simulink model "IEEE123bus_v2019b_Phasor_PI_ZIPload"  (R2019b)
settings: Solver=ode4  StartTime=0.0  StopTime=100  FixedStep=Ts  MaxStep=1e-4  RelTol=1e-3
InitFcn:
  | a=1; % Loading Factor
  | Ts=0.1;% For Delay Blocks in Voltage Regulator Controls
  | % phase to sequence conversion of RXB matrices
  | c=1*exp(sqrt(-1)*(120*pi/180));
  | T=[1 1 1;1 c*c c;1 c c*c];
  | Tinv=1/3*[1 1 1;1 c c*c;1 c*c c];
  | 
  | % Simulation data for the IEEE 123 Node Test Feeder model
  | mi2km = 1.60934;%  miles to km conversion
  | ft2km = 0.0003048; % feet to km conversion
  | ms2F = 1*1e-6/(2*pi*60);% microsiemens to Farads conversion
  | 
  | %% Configuration 1
  | % Series Resitance and Reactance - ohm/mile
  | R_1 = [0.4576 0.1560 0.1535;0.1560 0.4666 0.1580;0.1535 0.1580 0.4615];
  | X_1 = [1.0780 0.5017 0.3849;0.5017 1.0482 0.4236;0.3849 0.4236 1.0651];
  | % charging susceptance - microsiemens/mile
  | B_1 = [5.6765 -1.8319 -0.6982;-1.8319 5.9809 -1.1645;-0.6982 -1.1645 5.3971];
  | 
  | R_1 = R_1/mi2km;
  | Rseq=Tinv*R_1*T;
  | R1_1=Rseq(2,2);R0_1=Rseq(1,1);
  | 
  | L_1 = (X_1/(2*pi*60))/mi2km;
  | Lseq=Tinv*L_1*T;
  | L1_1=Lseq(2,2);L0_1=Lseq(1,1);
  | 
  | C_1 =(B_1*ms2F)/mi2km;
  | Cseq=Tinv*C_1*T;
  | C1_1=Cseq(2,2);C0_1=Cseq(1,1);
  | %% Configuration 2 - series reactance - ohm/mile
  | R_2 = [0.4666 0.1580 0.1560;0.1580 0.4615 0.1535;0.1560 0.1535 0.4576];
  | X_2 = [1.0482 0.4236 0.5017;0.4236 1.0651 0.3849;0.5017 0.3849 1.0780];
  | % charging susceptance - microsiemens/mile
  | B_2 = [5.9809 -1.1645 -1.8319;-1.1645 5.3971 -0.6982;-1.8319 -0.6982 5.6765];
  | 
  | R_2 = R_2/mi2km;
  | Rseq=Tinv*R_2*T;
  | R1_2=Rseq(2,2);R0_2=Rseq(1,1);
  | 
  | L_2 = (X_2/(2*pi*60))/mi2km;
  | Lseq=Tinv*L_2*T;
  | L1_2=Lseq(2,2);L0_2=Lseq(1,1);
  | 
  | C_2 =(B_2*ms2F)/mi2km;
  | Cseq=Tinv*C_2*T;
  | C1_2=Cseq(2,2);C0_2=Cseq(1,1);
  | %% Configuration 3 - series reactance - ohm/mile
  | R_3 = [0.4615 0.1535 0.1580;0.1535 0.4576 0.1560;0.1580 0.1560 0.4666];
  | X_3 = [1.0651 0.3849 0.4236;0.3849 1.0780 0.5017;0.4236 0.5017 1.0482];
  | % charging susceptance - microsiemens/mile
  | B_3 = [5.3971 -0.6982 -1.1645;-0.6982 5.6765 -1.8319; -1.1645 -1.8319 5.9809];
  | 
  | R_3 = R_3/mi2km;
  | Rseq=Tinv*R_3*T;
  | R1_3=Rseq(2,2);R0_3=Rseq(1,1);
  | 
  | L_3 = (X_3/(2*pi*60))/mi2km;
  | Lseq=Tinv*L_3*T;
  | L1_3=Lseq(2,2);L0_3=Lseq(1,1);
  | 
  | C_3 =(B_3*ms2F)/mi2km;
  | Cseq=Tinv*C_3*T;
  | C1_3=Cseq(2,2);C0_3=Cseq(1,1);
  | %% Configuration 4 - series reactance - ohm/mile
  | R_4 = [0.4615 0.1580 0.1535;0.1580 0.4666 0.1560;0.1535 0.1560 0.4576];
  | X_4 = [1.0651 0.4236 0.3849;0.4236 1.0482 0.5017;0.3849 0.5017 1.0780];
  | % charging susceptance - microsiemens/mile
  | B_4 = [5.3971 -1.1645 -0.6982;-1.1645 5.9809 -1.8319;-0.6982 -1.8319 5.6765];
  | 
  | R_4 = R_4/mi2km;
  | Rseq=Tinv*R_4*T;
  | R1_4=Rseq(2,2);R0_4=Rseq(1,1);
  | 
  | L_4 = (X_4/(2*pi*60))/mi2km;
  | Lseq=Tinv*L_4*T;
  | L1_4=Lseq(2,2);L0_4=Lseq(1,1);
  | 
  | C_4 =(B_4*ms2F)/mi2km;
  | Cseq=Tinv*C_4*T;
  | C1_4=Cseq(2,2);C0_4=Cseq(1,1);
  | %% Configuration 5 - series reactance - ohm/mile
  | R_5 = [0.4666 0.1560 0.1580;0.1560 0.4576 0.1535;0.1580 0.1535 0.4615];
  | X_5 = [1.0482 0.5017 0.4236;0.5017 1.0780 0.3849;0.4236 0.3849 1.0651];
  | % charging susceptance - microsiemens/mile
  | B_5 = [5.9809 -1.8319 -1.1645;-1.8319 5.6765 -0.6982;-1.1645 -0.6982 5.3971];
  | 
  | R_5 = R_5/mi2km;
  | Rseq=Tinv*R_5*T;
  | R1_5=Rseq(2,2);R0_5=Rseq(1,1);
  | 
  | L_5 = (X_5/(2*pi*60))/mi2km;
  | Lseq=Tinv*L_5*T;
  | L1_5=Lseq(2,2);L0_5=Lseq(1,1);
  | 
  | C_5 =(B_5*ms2F)/mi2km;
  | Cseq=Tinv*C_5*T;
  | C1_5=Cseq(2,2);C0_5=Cseq(1,1);
  | %% Configuration 6 - series reactance - ohm/mile
  | R_6 = [0.4576 0.1535 0.1560;0.1535 0.4615 0.1580;0.1560 0.1580 0.4666];
  | X_6 = [1.0780 0.3849 0.5017;0.3849 1.0651 0.4236;0.5017 0.4236 1.0482];
  | % charging susceptance - microsiemens/mile
  | B_6 = [5.6765 -0.6982 -1.8319;-0.6982 5.3971 -1.1645;-1.8319 -1.1645 5.9809];
  | 
  | R_6 = R_6/mi2km;
  | Rseq=Tinv*R_6*T;
  | R1_6=Rseq(2,2);R0_6=Rseq(1,1);
  | 
  | L_6 = (X_6/(2*pi*60))/mi2km;
  | Lseq=Tinv*L_6*T;
  | L1_6=Lseq(2,2);L0_6=Lseq(1,1);
  | 
  | C_6 =(B_6*ms2F)/mi2km;
  | Cseq=Tinv*C_6*T;
  | C1_6=Cseq(2,2);C0_6=Cseq(1,1);
  | %% Configuration 7 - series reactance - ohm/mile
  | R_7 = [0.4576 0.0000 0.1535;0.0000 0.0000 0.0000;0.1535 0.0000 0.4615];
  | X_7 = [1.0780 0.0000 0.3849;0.0000 0.0000 0.0000;0.3849 0.0000 1.0651];
  | % charging susceptance - microsiemens/mile
  | B_7 = [5.1154 0.0000 -1.0549;0.0000 0.0000 0.0000;-1.0549 0.0000 5.1704];
  | 
  | R_7 = R_7/mi2km;
  | Rseq=Tinv*R_7*T;
  | R1_7=Rseq(2,2);R0_7=Rseq(1,1);
  | 
  | L_7 = (X_7/(2*pi*60))/mi2km;
  | Lseq=Tinv*L_7*T;
  | L1_7=Lseq(2,2);L0_7=Lseq(1,1);
  | 
  | C_7 =(B_7*ms2F)/mi2km;
  | Cseq=Tinv*C_7*T;
  | C1_7=Cseq(2,2);C0_7=Cseq(1,1);
  | %% Configuration 8 - series reactance - ohm/mile
  | R_8 = [0.4576 0.1535 0.0000;0.1535 0.4615 0.0000;0.0000 0.0000 0.0000];
  | X_8 = [1.0780 0.3849 0.0000;0.3849 1.0651 0.0000;0.0000 0.0000 0.0000];
  | % charging susceptance - microsiemens/mile
  | B_8 = [5.1154 -1.0549 0.0000;-1.0549 5.1704 0.0000;0.0000 0.0000 0.0000];
  | 
  | R_8 = R_8/mi2km;
  | Rseq=Tinv*R_8*T;
  | R1_8=Rseq(2,2);R0_8=Rseq(1,1);
  | 
  | L_8 = (X_8/(2*pi*60))/mi2km;
  | Lseq=Tinv*L_8*T;
  | L1_8=Lseq(2,2);L0_8=Lseq(1,1);
  | 
  | C_8 =(B_8*ms2F)/mi2km;
  | Cseq=Tinv*C_8*T;
  | C1_8=Cseq(2,2);C0_8=Cseq(1,1);
  | %% Configuration 9 - series reactance - ohm/mile
  | R_9 = [1.3292 0 0;0 0 0;0 0 0];
  | X_9 = [1.3475 0 0;0 0 0;0 0 0];
  | % charging susceptance - microsiemens/mile
  | B_9 = [4.5193 0 0;0 0 0;0 0 0];
  | 
  | R_9 = R_9/mi2km;
  | Rseq=Tinv*R_9*T;
  | R1_9=Rseq(2,2);R0_9=Rseq(1,1);
  | 
  | L_9 = (X_9/(2*pi*60))/mi2km;
  | Lseq=Tinv*L_9*T;
  | L1_9=Lseq(2,2);L0_9=Lseq(1,1);
  | 
  | C_9 =(B_9*ms2F)/mi2km;
  | Cseq=Tinv*C_9*T;
  | C1_9=Cseq(2,2);C0_9=Cseq(1,1);
  | %% Configuration 10- series reactance - ohm/mile
  | R_10 = [0 0 0;0 1.3292 0;0 0 0];
  | X_10 = [0 0 0;0 1.3475 0;0 0 0];
  | % charging susceptance - microsiemens/mile
  | B_10 = [0 0 0;0 4.5193 0;0 0 0];
  | 
  | R_10 = R_10/mi2km;
  | Rseq=Tinv*R_10*T;
  | R1_10=Rseq(2,2);R0_10=Rseq(1,1);
  | 
  | L_10 = (X_10/(2*pi*60))/mi2km;
  | Lseq=Tinv*L_10*T;
  | L1_10=Lseq(2,2);L0_10=Lseq(1,1);
  | 
  | C_10 =(B_10*ms2F)/mi2km;
  | Cseq=Tinv*C_10*T;
  | C1_10=Cseq(2,2);C0_10=Cseq(1,1);
  | %% Configuration 11 - series reactance - ohm/mile
  | R_11 = [0 0 0;0 0 0;0 0 1.3292];
  | X_11 = [0 0 0;0 0 0;0 0 1.3475];
  | % charging susceptance - microsiemens/mile
  | B_11 = [0 0 0;0 0 0;0 0 4.5193];
  | 
  | R_11 = R_11/mi2km;
  | Rseq=Tinv*R_11*T;
  | R1_11=Rseq(2,2);R0_11=Rseq(1,1);
  | 
  | L_11 = (X_11/(2*pi*60))/mi2km;
  | Lseq=Tinv*L_11*T;
  | L1_11=Lseq(2,2);L0_11=Lseq(1,1);
  | 
  | C_11 =(B_11*ms2F)/mi2km;
  | Cseq=Tinv*C_11*T;
  | C1_11=Cseq(2,2);C0_11=Cseq(1,1);
  | %% Configuration 12 - series reactance - ohm/mile
  | R_12 = [1.5209 0.5198 0.4924;0.5198 1.5329 0.5198;0.4924 0.5198 1.5209];
  | X_12 = [0.7521 0.2775 0.2157;0.2775 0.7162 0.2775;0.2157 0.2775 0.7521];
  | % charging susceptance - microsiemens/mile
  | B_12 = [67.2242 0.0000 0.0000;0.0000 67.2242 0.0000;0.0000 0.0000 67.2242];
  | 
  | R_12 = R_12/mi2km;
  | Rseq=Tinv*R_12*T;
  | R1_12=Rseq(2,2);R0_12=Rseq(1,1);
  | 
  | L_12 = (X_12/(2*pi*60))/mi2km;
  | Lseq=Tinv*L_12*T;
  | L1_12=Lseq(2,2);L0_12=Lseq(1,1);
  | 
  | C_12 =(B_12*ms2F)/mi2km;
  | Cseq=Tinv*C_12*T;
  | C1_12=Cseq(2,2);C0_12=Cseq(1,1);
undefined symbols (not defined in the file or in its folder): D1, Delta, find_system, j
libraries: powerlib x974, powerlib_meascontrol x31
(part 1 of 13)
settings Model: ARTEMISmethode_block_infos=$$__separator__$$pi123variableloadwith3PV/ARTEMIS Guide$$__separator__$$  Creator=Arun  LastModifiedBy=USARSUR
settings DataIOCC: ReturnWorkspaceOutputs=off
settings DebuggingCC: UnconnectedInputMsg=none  UnconnectedOutputMsg=none  UnconnectedLineMsg=none  ArithmeticOperatorsInVariantConditions=warning
settings SFSimCC: SimUseLocalCustomCode=off  CustomCodeUndefinedFunction=UseInterfaceOnly
settings RTWCC: RTWUseLocalCustomCode=off
settings CodeAppCC: StateflowObjectComments=on
settings SimscapeCC: SimscapeNormalizeSystem=off

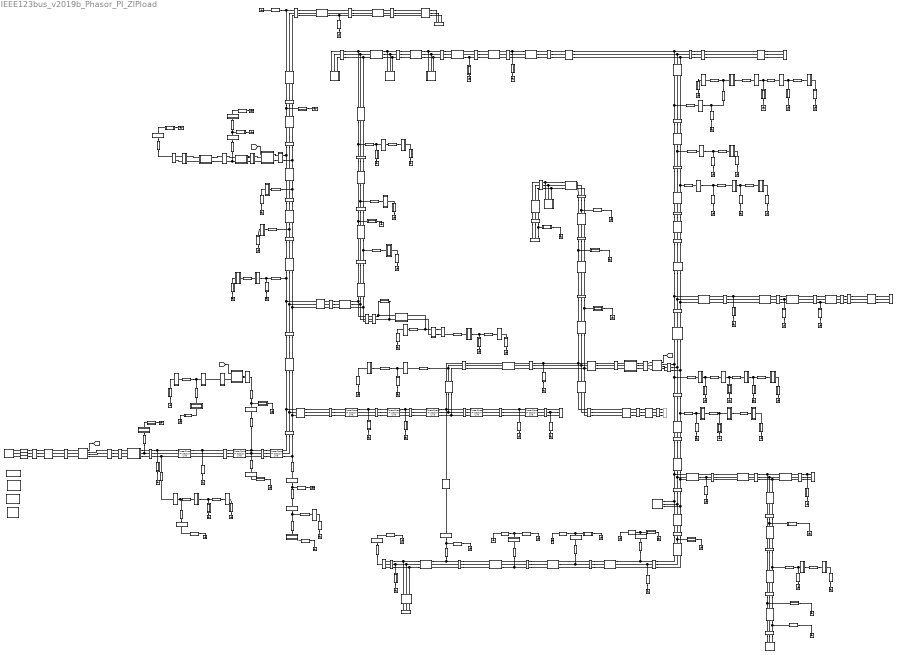
== system IEEE123bus_v2019b_Phasor_PI_ZIPload ==
  note: Please consider citing following papers if the model was useful for your research
      |
      | A. Suresh, R. Bisht and S. Kamalasadan, "A Coordinated Control Architecture With Inverter-Based Resources and Legacy
      | Controllers of Power Distribution System for Voltage Profile Balance," in IEEE Transactions on Industry Applications, vol. 58,
      | no. 5, pp. 6701-6712, Sept.-Oct. 2022, doi: 10.1109/TIA.2022.3183030.
      |
      | A. Suresh, R. Bisht and S. Kamalasadan, "ADMM Based LQR for Voltage Regulation Using Distributed Energy Resources,"
      | 2020 IEEE International Conference on Power Electronics, Drives and Energy Systems (PEDES), 2020, pp. 1-6,
      | doi: 10.1109/PEDES49360.2020.9379625.
  note: Model Developed by
      | Arun Suresh, Dr. Sukumar Kamalasadan,
      | University of North Carolina, Charlotte
  1 : powerlib/Measurements/Three-Phase V-I Measurement  VoltageMeasurement=phase-to-ground  SetLabelV=on  LabelV=V1  Vpu=off  VpuLL=off  CurrentMeasurement=no  SetLabelI=on  LabelI=I800  Ipu=off  Pbase=100e6  Vbase=24900  OutputType=Complex  PhasorSimulation=on  PSBequivalent=0
      settings: SourceProductName=Simscape Electrical
  1 Y PQ : Subsystem  mask(Single Phase ZIP Load){Vnom=1.0*2401.78, fnom=60, Pnom=40e3*a, Qnom=20e3*a, LoadType=constant P, Vlim=0.7}
      mask prompts: Vnom "Nominal Voltage Vn (Vrms)"; fnom "Nominal Frequency fn (Hz)"; Pnom "Nominal Active power (W)"; Qnom "Nominal Reactive power (VAR)"; LoadType "Load Type"; Vlim "Minimum voltage (pu)"
      mask help:
      | Notes:
      | Single Phase ZIP load model which gets converted to constant Z type if the voltage becomes lower than the Minimum Voltage.
      mask TypeOptions LoadType: Constant Z | constant I | constant P
      mask DialogControl ParameterTabVar0 Prompt: Parameters
      mask DialogControl ParameterTabVar1 Prompt: Type
      mask Display:
      | color('red');
      | A=[-210,-180,-170,-160,-147,-140,-130,-120,-110,-80,-50,-49,-45,-39,-33,-26,-21,-18,-17,-19,-22,-22,-26,-27,-25,-22,-16,-9,-3,2,6,6,4,1,1,-3,-4,-2,2,7,14,20,26,29,30,28,24,24,21,20,21,25,31,37,44,49,50,50,80];
      | B=[-41.5,-41.5,-63,-20,-63,-20,-63,-20,-41.5,-41.5,-41.5,-34,-26,-21,-20,-22,-28,-37,-47,-57,-63,-63,-54,-44,-34,-26,-21,-20,-22,-28,-37,-47,-57,-63,-63,-54,-44,-34,-26,-21,-20,-22,-28,-37,-47,-57,-63,-63,-54,-44,-34,-26,-21,-20,-22,-28,-37,-41.50,-41.5];
      | plot(A,B);
      | color('black');
      | port_label('LConn', 1, '+')
  1-2 10 : powerlib/Elements/Pi Section Line  LConnTagsString=__new0  RConnTagsString=__new0  Frequency=60  Resistance=R1_10  Inductance=L1_10  Capacitance=C1_10  Length=175*ft2km  PiSections=1  Measurements=None
      settings: AttributesFormatString=\n  SourceProductName=Simscape Electrical  SourceProductBaseCode=PS
  1-3 11 : powerlib/Elements/Pi Section Line  LConnTagsString=__new0  RConnTagsString=__new0  Frequency=60  Resistance=R1_11  Inductance=L1_11  Capacitance=C1_11  Length=250*ft2km  PiSections=1  Measurements=None
      settings: AttributesFormatString=\n  SourceProductName=Simscape Electrical  SourceProductBaseCode=PS
  1-7 1 : powerlib/Elements/Three-Phase PI Section Line  LConnTagsString=a|b|c  RConnTagsString=A|B|C  Frequency=60  Resistances=[R1_1 R0_1]  Inductances=[L1_1 L0_1]  Capacitances=[C1_1 C0_1]  Length=300*ft2km
      settings: SourceProductName=Simscape Electrical
  10 : Subsystem
  10 Y I : Subsystem  mask(Single Phase ZIP Load){Vnom=1.0*2401.78, fnom=60, Pnom=20e3*a, Qnom=10e3*a, LoadType=constant I, Vlim=0.7}
      mask prompts: Vnom "Nominal Voltage Vn (Vrms)"; fnom "Nominal Frequency fn (Hz)"; Pnom "Nominal Active power (W)"; Qnom "Nominal Reactive power (VAR)"; LoadType "Load Type"; Vlim "Minimum voltage (pu)"
      mask help:
      | Notes:
      | Single Phase ZIP load model which gets converted to constant Z type if the voltage becomes lower than the Minimum Voltage.
      mask TypeOptions LoadType: Constant Z | constant I | constant P
      mask DialogControl ParameterTabVar0 Prompt: Parameters
      mask DialogControl ParameterTabVar1 Prompt: Type
      mask Display:
      | color('red');
      | A=[-210,-180,-170,-160,-147,-140,-130,-120,-110,-80,-50,-49,-45,-39,-33,-26,-21,-18,-17,-19,-22,-22,-26,-27,-25,-22,-16,-9,-3,2,6,6,4,1,1,-3,-4,-2,2,7,14,20,26,29,30,28,24,24,21,20,21,25,31,37,44,49,50,50,80];
      | B=[-41.5,-41.5,-63,-20,-63,-20,-63,-20,-41.5,-41.5,-41.5,-34,-26,-21,-20,-22,-28,-37,-47,-57,-63,-63,-54,-44,-34,-26,-21,-20,-22,-28,-37,-47,-57,-63,-63,-54,-44,-34,-26,-21,-20,-22,-28,-37,-47,-57,-63,-63,-54,-44,-34,-26,-21,-20,-22,-28,-37,-41.50,-41.5];
      | plot(A,B);
      | color('black');
      | port_label('LConn', 1, '+')
  100 : powerlib/Measurements/Three-Phase V-I Measurement  VoltageMeasurement=phase-to-ground  SetLabelV=on  LabelV=V100  Vpu=off  VpuLL=off  CurrentMeasurement=no  SetLabelI=on  LabelI=I65  Ipu=off  Pbase=100e6  Vbase=24900  OutputType=Complex  PhasorSimulation=on  PSBequivalent=0
      settings: SourceProductName=Simscape Electrical
  100 Y Z : Subsystem  mask(Single Phase ZIP Load){Vnom=1.0*2401.78, fnom=60, Pnom=40e3*a, Qnom=20e3*a, LoadType=Constant Z, Vlim=0.7}
      mask prompts: Vnom "Nominal Voltage Vn (Vrms)"; fnom "Nominal Frequency fn (Hz)"; Pnom "Nominal Active power (W)"; Qnom "Nominal Reactive power (VAR)"; LoadType "Load Type"; Vlim "Minimum voltage (pu)"
      mask help:
      | Notes:
      | Single Phase ZIP load model which gets converted to constant Z type if the voltage becomes lower than the Minimum Voltage.
      mask TypeOptions LoadType: Constant Z | constant I | constant P
      mask DialogControl ParameterTabVar0 Prompt: Parameters
      mask DialogControl ParameterTabVar1 Prompt: Type
      mask Display:
      | color('red');
      | A=[-210,-180,-170,-160,-147,-140,-130,-120,-110,-80,-50,-49,-45,-39,-33,-26,-21,-18,-17,-19,-22,-22,-26,-27,-25,-22,-16,-9,-3,2,6,6,4,1,1,-3,-4,-2,2,7,14,20,26,29,30,28,24,24,21,20,21,25,31,37,44,49,50,50,80];
      | B=[-41.5,-41.5,-63,-20,-63,-20,-63,-20,-41.5,-41.5,-41.5,-34,-26,-21,-20,-22,-28,-37,-47,-57,-63,-63,-54,-44,-34,-26,-21,-20,-22,-28,-37,-47,-57,-63,-63,-54,-44,-34,-26,-21,-20,-22,-28,-37,-47,-57,-63,-63,-54,-44,-34,-26,-21,-20,-22,-28,-37,-41.50,-41.5];
      | plot(A,B);
      | color('black');
      | port_label('LConn', 1, '+')
  100-450 3 : powerlib/Elements/Three-Phase PI Section Line  LConnTagsString=a|b|c  RConnTagsString=A|B|C  Frequency=60  Resistances=[R1_3 R0_3]  Inductances=[L1_3 L0_3]  Capacitances=[C1_3 C0_3]  Length=800*ft2km
      settings: SourceProductName=Simscape Electrical
  101 : powerlib/Measurements/Three-Phase V-I Measurement  VoltageMeasurement=phase-to-ground  SetLabelV=on  LabelV=V101  Vpu=off  VpuLL=off  CurrentMeasurement=no  SetLabelI=on  LabelI=I65  Ipu=off  Pbase=100e6  Vbase=24900  OutputType=Complex  PhasorSimulation=on  PSBequivalent=0
      settings: SourceProductName=Simscape Electrical
  101-102 11 : powerlib/Elements/Pi Section Line  LConnTagsString=__new0  RConnTagsString=__new0  Frequency=60  Resistance=R1_11  Inductance=L1_11  Capacitance=C1_11  Length=225*ft2km  PiSections=1  Measurements=None
      settings: AttributesFormatString=\n  SourceProductName=Simscape Electrical  SourceProductBaseCode=PS
  101-105 3 : powerlib/Elements/Three-Phase PI Section Line  LConnTagsString=a|b|c  RConnTagsString=A|B|C  Frequency=60  Resistances=[R1_3 R0_3]  Inductances=[L1_3 L0_3]  Capacitances=[C1_3 C0_3]  Length=275*ft2km
      settings: SourceProductName=Simscape Electrical
  102 : Subsystem
  102 Y PQ : Subsystem  mask(Single Phase ZIP Load){Vnom=1.0*2401.78, fnom=60, Pnom=20e3*a, Qnom=10e3*a, LoadType=constant P, Vlim=0.7}
      mask prompts: Vnom "Nominal Voltage Vn (Vrms)"; fnom "Nominal Frequency fn (Hz)"; Pnom "Nominal Active power (W)"; Qnom "Nominal Reactive power (VAR)"; LoadType "Load Type"; Vlim "Minimum voltage (pu)"
      mask help:
      | Notes:
      | Single Phase ZIP load model which gets converted to constant Z type if the voltage becomes lower than the Minimum Voltage.
      mask TypeOptions LoadType: Constant Z | constant I | constant P
      mask DialogControl ParameterTabVar0 Prompt: Parameters
      mask DialogControl ParameterTabVar1 Prompt: Type
      mask Display:
      | color('red');
      | A=[-210,-180,-170,-160,-147,-140,-130,-120,-110,-80,-50,-49,-45,-39,-33,-26,-21,-18,-17,-19,-22,-22,-26,-27,-25,-22,-16,-9,-3,2,6,6,4,1,1,-3,-4,-2,2,7,14,20,26,29,30,28,24,24,21,20,21,25,31,37,44,49,50,50,80];
      | B=[-41.5,-41.5,-63,-20,-63,-20,-63,-20,-41.5,-41.5,-41.5,-34,-26,-21,-20,-22,-28,-37,-47,-57,-63,-63,-54,-44,-34,-26,-21,-20,-22,-28,-37,-47,-57,-63,-63,-54,-44,-34,-26,-21,-20,-22,-28,-37,-47,-57,-63,-63,-54,-44,-34,-26,-21,-20,-22,-28,-37,-41.50,-41.5];
      | plot(A,B);
      | color('black');
      | port_label('LConn', 1, '+')
  102-103 11 : powerlib/Elements/Pi Section Line  LConnTagsString=__new0  RConnTagsString=__new0  Frequency=60  Resistance=R1_11  Inductance=L1_11  Capacitance=C1_11  Length=325*ft2km  PiSections=1  Measurements=None
      settings: AttributesFormatString=\n  SourceProductName=Simscape Electrical  SourceProductBaseCode=PS
  103 : Subsystem
  103 Y PQ : Subsystem  mask(Single Phase ZIP Load){Vnom=1.0*2401.78, fnom=60, Pnom=40e3*a, Qnom=20e3*a, LoadType=constant P, Vlim=0.7}
      mask prompts: Vnom "Nominal Voltage Vn (Vrms)"; fnom "Nominal Frequency fn (Hz)"; Pnom "Nominal Active power (W)"; Qnom "Nominal Reactive power (VAR)"; LoadType "Load Type"; Vlim "Minimum voltage (pu)"
      mask help:
      | Notes:
      | Single Phase ZIP load model which gets converted to constant Z type if the voltage becomes lower than the Minimum Voltage.
      mask TypeOptions LoadType: Constant Z | constant I | constant P
      mask DialogControl ParameterTabVar0 Prompt: Parameters
      mask DialogControl ParameterTabVar1 Prompt: Type
      mask Display:
      | color('red');
      | A=[-210,-180,-170,-160,-147,-140,-130,-120,-110,-80,-50,-49,-45,-39,-33,-26,-21,-18,-17,-19,-22,-22,-26,-27,-25,-22,-16,-9,-3,2,6,6,4,1,1,-3,-4,-2,2,7,14,20,26,29,30,28,24,24,21,20,21,25,31,37,44,49,50,50,80];
      | B=[-41.5,-41.5,-63,-20,-63,-20,-63,-20,-41.5,-41.5,-41.5,-34,-26,-21,-20,-22,-28,-37,-47,-57,-63,-63,-54,-44,-34,-26,-21,-20,-22,-28,-37,-47,-57,-63,-63,-54,-44,-34,-26,-21,-20,-22,-28,-37,-47,-57,-63,-63,-54,-44,-34,-26,-21,-20,-22,-28,-37,-41.50,-41.5];
      | plot(A,B);
      | color('black');
      | port_label('LConn', 1, '+')
  103-104 11 : powerlib/Elements/Pi Section Line  LConnTagsString=__new0  RConnTagsString=__new0  Frequency=60  Resistance=R1_11  Inductance=L1_11  Capacitance=C1_11  Length=700*ft2km  PiSections=1  Measurements=None
      settings: AttributesFormatString=\n  SourceProductName=Simscape Electrical  SourceProductBaseCode=PS
  104 : Subsystem
  104 Y PQ : Subsystem  mask(Single Phase ZIP Load){Vnom=1.0*2401.78, fnom=60, Pnom=40e3*a, Qnom=20e3*a, LoadType=constant P, Vlim=0.7}
      mask prompts: Vnom "Nominal Voltage Vn (Vrms)"; fnom "Nominal Frequency fn (Hz)"; Pnom "Nominal Active power (W)"; Qnom "Nominal Reactive power (VAR)"; LoadType "Load Type"; Vlim "Minimum voltage (pu)"
      mask help:
      | Notes:
      | Single Phase ZIP load model which gets converted to constant Z type if the voltage becomes lower than the Minimum Voltage.
      mask TypeOptions LoadType: Constant Z | constant I | constant P
      mask DialogControl ParameterTabVar0 Prompt: Parameters
      mask DialogControl ParameterTabVar1 Prompt: Type
      mask Display:
      | color('red');
      | A=[-210,-180,-170,-160,-147,-140,-130,-120,-110,-80,-50,-49,-45,-39,-33,-26,-21,-18,-17,-19,-22,-22,-26,-27,-25,-22,-16,-9,-3,2,6,6,4,1,1,-3,-4,-2,2,7,14,20,26,29,30,28,24,24,21,20,21,25,31,37,44,49,50,50,80];
      | B=[-41.5,-41.5,-63,-20,-63,-20,-63,-20,-41.5,-41.5,-41.5,-34,-26,-21,-20,-22,-28,-37,-47,-57,-63,-63,-54,-44,-34,-26,-21,-20,-22,-28,-37,-47,-57,-63,-63,-54,-44,-34,-26,-21,-20,-22,-28,-37,-47,-57,-63,-63,-54,-44,-34,-26,-21,-20,-22,-28,-37,-41.50,-41.5];
      | plot(A,B);
      | color('black');
      | port_label('LConn', 1, '+')
  105 : powerlib/Measurements/Three-Phase V-I Measurement  VoltageMeasurement=phase-to-ground  SetLabelV=on  LabelV=V105  Vpu=off  VpuLL=off  CurrentMeasurement=no  SetLabelI=on  LabelI=I65  Ipu=off  Pbase=100e6  Vbase=24900  OutputType=Complex  PhasorSimulation=on  PSBequivalent=0
      settings: SourceProductName=Simscape Electrical
  105-106 10 : powerlib/Elements/Pi Section Line  LConnTagsString=__new0  RConnTagsString=__new0  Frequency=60  Resistance=R1_10  Inductance=L1_10  Capacitance=C1_10  Length=225*ft2km  PiSections=1  Measurements=None
      settings: AttributesFormatString=\n  SourceProductName=Simscape Electrical  SourceProductBaseCode=PS
  105-108 3 : powerlib/Elements/Three-Phase PI Section Line  LConnTagsString=a|b|c  RConnTagsString=A|B|C  Frequency=60  Resistances=[R1_3 R0_3]  Inductances=[L1_3 L0_3]  Capacitances=[C1_3 C0_3]  Length=325*ft2km
      settings: SourceProductName=Simscape Electrical
  106 : Subsystem
  106 Y PQ : Subsystem  mask(Single Phase ZIP Load){Vnom=1.0*2401.78, fnom=60, Pnom=40e3*a, Qnom=20e3*a, LoadType=constant P, Vlim=0.7}
      mask prompts: Vnom "Nominal Voltage Vn (Vrms)"; fnom "Nominal Frequency fn (Hz)"; Pnom "Nominal Active power (W)"; Qnom "Nominal Reactive power (VAR)"; LoadType "Load Type"; Vlim "Minimum voltage (pu)"
      mask help:
      | Notes:
      | Single Phase ZIP load model which gets converted to constant Z type if the voltage becomes lower than the Minimum Voltage.
      mask TypeOptions LoadType: Constant Z | constant I | constant P
      mask DialogControl ParameterTabVar0 Prompt: Parameters
      mask DialogControl ParameterTabVar1 Prompt: Type
      mask Display:
      | color('red');
      | A=[-210,-180,-170,-160,-147,-140,-130,-120,-110,-80,-50,-49,-45,-39,-33,-26,-21,-18,-17,-19,-22,-22,-26,-27,-25,-22,-16,-9,-3,2,6,6,4,1,1,-3,-4,-2,2,7,14,20,26,29,30,28,24,24,21,20,21,25,31,37,44,49,50,50,80];
      | B=[-41.5,-41.5,-63,-20,-63,-20,-63,-20,-41.5,-41.5,-41.5,-34,-26,-21,-20,-22,-28,-37,-47,-57,-63,-63,-54,-44,-34,-26,-21,-20,-22,-28,-37,-47,-57,-63,-63,-54,-44,-34,-26,-21,-20,-22,-28,-37,-47,-57,-63,-63,-54,-44,-34,-26,-21,-20,-22,-28,-37,-41.50,-41.5];
      | plot(A,B);
      | color('black');
      | port_label('LConn', 1, '+')
  106-107 10 : powerlib/Elements/Pi Section Line  LConnTagsString=__new0  RConnTagsString=__new0  Frequency=60  Resistance=R1_10  Inductance=L1_10  Capacitance=C1_10  Length=575*ft2km  PiSections=1  Measurements=None
      settings: AttributesFormatString=\n  SourceProductName=Simscape Electrical  SourceProductBaseCode=PS
  107 : Subsystem
  107 Y PQ : Subsystem  mask(Single Phase ZIP Load){Vnom=1.0*2401.78, fnom=60, Pnom=40e3*a, Qnom=20e3*a, LoadType=constant P, Vlim=0.7}
      mask prompts: Vnom "Nominal Voltage Vn (Vrms)"; fnom "Nominal Frequency fn (Hz)"; Pnom "Nominal Active power (W)"; Qnom "Nominal Reactive power (VAR)"; LoadType "Load Type"; Vlim "Minimum voltage (pu)"
      mask help:
      | Notes:
      | Single Phase ZIP load model which gets converted to constant Z type if the voltage becomes lower than the Minimum Voltage.
      mask TypeOptions LoadType: Constant Z | constant I | constant P
      mask DialogControl ParameterTabVar0 Prompt: Parameters
      mask DialogControl ParameterTabVar1 Prompt: Type
      mask Display:
      | color('red');
      | A=[-210,-180,-170,-160,-147,-140,-130,-120,-110,-80,-50,-49,-45,-39,-33,-26,-21,-18,-17,-19,-22,-22,-26,-27,-25,-22,-16,-9,-3,2,6,6,4,1,1,-3,-4,-2,2,7,14,20,26,29,30,28,24,24,21,20,21,25,31,37,44,49,50,50,80];
      | B=[-41.5,-41.5,-63,-20,-63,-20,-63,-20,-41.5,-41.5,-41.5,-34,-26,-21,-20,-22,-28,-37,-47,-57,-63,-63,-54,-44,-34,-26,-21,-20,-22,-28,-37,-47,-57,-63,-63,-54,-44,-34,-26,-21,-20,-22,-28,-37,-47,-57,-63,-63,-54,-44,-34,-26,-21,-20,-22,-28,-37,-41.50,-41.5];
      | plot(A,B);
      | color('black');
      | port_label('LConn', 1, '+')
  108 : powerlib/Measurements/Three-Phase V-I Measurement  VoltageMeasurement=phase-to-ground  SetLabelV=on  LabelV=V108  Vpu=off  VpuLL=off  CurrentMeasurement=no  SetLabelI=on  LabelI=I65  Ipu=off  Pbase=100e6  Vbase=24900  OutputType=Complex  PhasorSimulation=on  PSBequivalent=0
      settings: SourceProductName=Simscape Electrical
  108-109 9 : powerlib/Elements/Pi Section Line  LConnTagsString=__new0  RConnTagsString=__new0  Frequency=60  Resistance=R1_9  Inductance=L1_9  Capacitance=C1_9  Length=450*ft2km  PiSections=1  Measurements=None
      settings: AttributesFormatString=\n  SourceProductName=Simscape Electrical  SourceProductBaseCode=PS
  108-300 3 : powerlib/Elements/Three-Phase PI Section Line  LConnTagsString=a|b|c  RConnTagsString=A|B|C  Frequency=60  Resistances=[R1_3 R0_3]  Inductances=[L1_3 L0_3]  Capacitances=[C1_3 C0_3]  Length=1000*ft2km
      settings: SourceProductName=Simscape Electrical
  109 : Subsystem
  109 Y PQ : Subsystem  mask(Single Phase ZIP Load){Vnom=1.0*2401.78, fnom=60, Pnom=40e3*a, Qnom=20e3*a, LoadType=constant P, Vlim=0.7}
      mask prompts: Vnom "Nominal Voltage Vn (Vrms)"; fnom "Nominal Frequency fn (Hz)"; Pnom "Nominal Active power (W)"; Qnom "Nominal Reactive power (VAR)"; LoadType "Load Type"; Vlim "Minimum voltage (pu)"
      mask help:
      | Notes:
      | Single Phase ZIP load model which gets converted to constant Z type if the voltage becomes lower than the Minimum Voltage.
      mask TypeOptions LoadType: Constant Z | constant I | constant P
      mask DialogControl ParameterTabVar0 Prompt: Parameters
      mask DialogControl ParameterTabVar1 Prompt: Type
      mask Display:
      | color('red');
      | A=[-210,-180,-170,-160,-147,-140,-130,-120,-110,-80,-50,-49,-45,-39,-33,-26,-21,-18,-17,-19,-22,-22,-26,-27,-25,-22,-16,-9,-3,2,6,6,4,1,1,-3,-4,-2,2,7,14,20,26,29,30,28,24,24,21,20,21,25,31,37,44,49,50,50,80];
      | B=[-41.5,-41.5,-63,-20,-63,-20,-63,-20,-41.5,-41.5,-41.5,-34,-26,-21,-20,-22,-28,-37,-47,-57,-63,-63,-54,-44,-34,-26,-21,-20,-22,-28,-37,-47,-57,-63,-63,-54,-44,-34,-26,-21,-20,-22,-28,-37,-47,-57,-63,-63,-54,-44,-34,-26,-21,-20,-22,-28,-37,-41.50,-41.5];
      | plot(A,B);
      | color('black');
      | port_label('LConn', 1, '+')
  109-110 9 : powerlib/Elements/Pi Section Line  LConnTagsString=__new0  RConnTagsString=__new0  Frequency=60  Resistance=R1_9  Inductance=L1_9  Capacitance=C1_9  Length=300*ft2km  PiSections=1  Measurements=None
      settings: AttributesFormatString=\n  SourceProductName=Simscape Electrical  SourceProductBaseCode=PS
  11 : Subsystem
  11 Y Z : Subsystem  mask(Single Phase ZIP Load){Vnom=1.0*2401.78, fnom=60, Pnom=40e3*a, Qnom=20e3*a, LoadType=Constant Z, Vlim=0.7}
      mask prompts: Vnom "Nominal Voltage Vn (Vrms)"; fnom "Nominal Frequency fn (Hz)"; Pnom "Nominal Active power (W)"; Qnom "Nominal Reactive power (VAR)"; LoadType "Load Type"; Vlim "Minimum voltage (pu)"
      mask help:
      | Notes:
      | Single Phase ZIP load model which gets converted to constant Z type if the voltage becomes lower than the Minimum Voltage.
      mask TypeOptions LoadType: Constant Z | constant I | constant P
      mask DialogControl ParameterTabVar0 Prompt: Parameters
      mask DialogControl ParameterTabVar1 Prompt: Type
      mask Display:
      | color('red');
      | A=[-210,-180,-170,-160,-147,-140,-130,-120,-110,-80,-50,-49,-45,-39,-33,-26,-21,-18,-17,-19,-22,-22,-26,-27,-25,-22,-16,-9,-3,2,6,6,4,1,1,-3,-4,-2,2,7,14,20,26,29,30,28,24,24,21,20,21,25,31,37,44,49,50,50,80];
      | B=[-41.5,-41.5,-63,-20,-63,-20,-63,-20,-41.5,-41.5,-41.5,-34,-26,-21,-20,-22,-28,-37,-47,-57,-63,-63,-54,-44,-34,-26,-21,-20,-22,-28,-37,-47,-57,-63,-63,-54,-44,-34,-26,-21,-20,-22,-28,-37,-47,-57,-63,-63,-54,-44,-34,-26,-21,-20,-22,-28,-37,-41.50,-41.5];
      | plot(A,B);
      | color('black');
      | port_label('LConn', 1, '+')
  110 : Subsystem
  110-111 9 : powerlib/Elements/Pi Section Line  LConnTagsString=__new0  RConnTagsString=__new0  Frequency=60  Resistance=R1_9  Inductance=L1_9  Capacitance=C1_9  Length=575*ft2km  PiSections=1  Measurements=None
      settings: AttributesFormatString=\n  SourceProductName=Simscape Electrical  SourceProductBaseCode=PS
  110-112 9 : powerlib/Elements/Pi Section Line  LConnTagsString=__new0  RConnTagsString=__new0  Frequency=60  Resistance=R1_9  Inductance=L1_9  Capacitance=C1_9  Length=125*ft2km  PiSections=1  Measurements=None
      settings: AttributesFormatString=\n  SourceProductName=Simscape Electrical  SourceProductBaseCode=PS
  111 : Subsystem
  111 Y PQ : Subsystem  mask(Single Phase ZIP Load){Vnom=1.0*2401.78, fnom=60, Pnom=20e3*a, Qnom=10e3*a, LoadType=constant P, Vlim=0.7}
      mask prompts: Vnom "Nominal Voltage Vn (Vrms)"; fnom "Nominal Frequency fn (Hz)"; Pnom "Nominal Active power (W)"; Qnom "Nominal Reactive power (VAR)"; LoadType "Load Type"; Vlim "Minimum voltage (pu)"
      mask help:
      | Notes:
      | Single Phase ZIP load model which gets converted to constant Z type if the voltage becomes lower than the Minimum Voltage.
      mask TypeOptions LoadType: Constant Z | constant I | constant P
      mask DialogControl ParameterTabVar0 Prompt: Parameters
      mask DialogControl ParameterTabVar1 Prompt: Type
      mask Display:
      | color('red');
      | A=[-210,-180,-170,-160,-147,-140,-130,-120,-110,-80,-50,-49,-45,-39,-33,-26,-21,-18,-17,-19,-22,-22,-26,-27,-25,-22,-16,-9,-3,2,6,6,4,1,1,-3,-4,-2,2,7,14,20,26,29,30,28,24,24,21,20,21,25,31,37,44,49,50,50,80];
      | B=[-41.5,-41.5,-63,-20,-63,-20,-63,-20,-41.5,-41.5,-41.5,-34,-26,-21,-20,-22,-28,-37,-47,-57,-63,-63,-54,-44,-34,-26,-21,-20,-22,-28,-37,-47,-57,-63,-63,-54,-44,-34,-26,-21,-20,-22,-28,-37,-47,-57,-63,-63,-54,-44,-34,-26,-21,-20,-22,-28,-37,-41.50,-41.5];
      | plot(A,B);
      | color('black');
      | port_label('LConn', 1, '+')
  112 : Subsystem
  112 Y I : Subsystem  mask(Single Phase ZIP Load){Vnom=1.0*2401.78, fnom=60, Pnom=20e3*a, Qnom=10e3*a, LoadType=constant I, Vlim=0.7}
      mask prompts: Vnom "Nominal Voltage Vn (Vrms)"; fnom "Nominal Frequency fn (Hz)"; Pnom "Nominal Active power (W)"; Qnom "Nominal Reactive power (VAR)"; LoadType "Load Type"; Vlim "Minimum voltage (pu)"
      mask help:
      | Notes:
      | Single Phase ZIP load model which gets converted to constant Z type if the voltage becomes lower than the Minimum Voltage.
      mask TypeOptions LoadType: Constant Z | constant I | constant P
      mask DialogControl ParameterTabVar0 Prompt: Parameters
      mask DialogControl ParameterTabVar1 Prompt: Type
      mask Display:
      | color('red');
      | A=[-210,-180,-170,-160,-147,-140,-130,-120,-110,-80,-50,-49,-45,-39,-33,-26,-21,-18,-17,-19,-22,-22,-26,-27,-25,-22,-16,-9,-3,2,6,6,4,1,1,-3,-4,-2,2,7,14,20,26,29,30,28,24,24,21,20,21,25,31,37,44,49,50,50,80];
      | B=[-41.5,-41.5,-63,-20,-63,-20,-63,-20,-41.5,-41.5,-41.5,-34,-26,-21,-20,-22,-28,-37,-47,-57,-63,-63,-54,-44,-34,-26,-21,-20,-22,-28,-37,-47,-57,-63,-63,-54,-44,-34,-26,-21,-20,-22,-28,-37,-47,-57,-63,-63,-54,-44,-34,-26,-21,-20,-22,-28,-37,-41.50,-41.5];
      | plot(A,B);
      | color('black');
      | port_label('LConn', 1, '+')
  112-113 9 : powerlib/Elements/Pi Section Line  LConnTagsString=__new0  RConnTagsString=__new0  Frequency=60  Resistance=R1_9  Inductance=L1_9  Capacitance=C1_9  Length=525*ft2km  PiSections=1  Measurements=None
      settings: AttributesFormatString=\n  SourceProductName=Simscape Electrical  SourceProductBaseCode=PS
  113 : Subsystem
  113 Y Z : Subsystem  mask(Single Phase ZIP Load){Vnom=1.0*2401.78, fnom=60, Pnom=40e3*a, Qnom=20e3*a, LoadType=Constant Z, Vlim=0.7}
      mask prompts: Vnom "Nominal Voltage Vn (Vrms)"; fnom "Nominal Frequency fn (Hz)"; Pnom "Nominal Active power (W)"; Qnom "Nominal Reactive power (VAR)"; LoadType "Load Type"; Vlim "Minimum voltage (pu)"
      mask help:
      | Notes:
      | Single Phase ZIP load model which gets converted to constant Z type if the voltage becomes lower than the Minimum Voltage.
      mask TypeOptions LoadType: Constant Z | constant I | constant P
      mask DialogControl ParameterTabVar0 Prompt: Parameters
      mask DialogControl ParameterTabVar1 Prompt: Type
      mask Display:
      | color('red');
      | A=[-210,-180,-170,-160,-147,-140,-130,-120,-110,-80,-50,-49,-45,-39,-33,-26,-21,-18,-17,-19,-22,-22,-26,-27,-25,-22,-16,-9,-3,2,6,6,4,1,1,-3,-4,-2,2,7,14,20,26,29,30,28,24,24,21,20,21,25,31,37,44,49,50,50,80];
      | B=[-41.5,-41.5,-63,-20,-63,-20,-63,-20,-41.5,-41.5,-41.5,-34,-26,-21,-20,-22,-28,-37,-47,-57,-63,-63,-54,-44,-34,-26,-21,-20,-22,-28,-37,-47,-57,-63,-63,-54,-44,-34,-26,-21,-20,-22,-28,-37,-47,-57,-63,-63,-54,-44,-34,-26,-21,-20,-22,-28,-37,-41.50,-41.5];
      | plot(A,B);
      | color('black');
      | port_label('LConn', 1, '+')
  113-114 9 : powerlib/Elements/Pi Section Line  LConnTagsString=__new0  RConnTagsString=__new0  Frequency=60  Resistance=R1_9  Inductance=L1_9  Capacitance=C1_9  Length=325*ft2km  PiSections=1  Measurements=None
      settings: AttributesFormatString=\n  SourceProductName=Simscape Electrical  SourceProductBaseCode=PS
  114 : Subsystem
  114 Y PQ : Subsystem  mask(Single Phase ZIP Load){Vnom=1.0*2401.78, fnom=60, Pnom=20e3*a, Qnom=10e3*a, LoadType=constant P, Vlim=0.7}
      mask prompts: Vnom "Nominal Voltage Vn (Vrms)"; fnom "Nominal Frequency fn (Hz)"; Pnom "Nominal Active power (W)"; Qnom "Nominal Reactive power (VAR)"; LoadType "Load Type"; Vlim "Minimum voltage (pu)"
      mask help:
      | Notes:
      | Single Phase ZIP load model which gets converted to constant Z type if the voltage becomes lower than the Minimum Voltage.
      mask TypeOptions LoadType: Constant Z | constant I | constant P
      mask DialogControl ParameterTabVar0 Prompt: Parameters
      mask DialogControl ParameterTabVar1 Prompt: Type
      mask Display:
      | color('red');
      | A=[-210,-180,-170,-160,-147,-140,-130,-120,-110,-80,-50,-49,-45,-39,-33,-26,-21,-18,-17,-19,-22,-22,-26,-27,-25,-22,-16,-9,-3,2,6,6,4,1,1,-3,-4,-2,2,7,14,20,26,29,30,28,24,24,21,20,21,25,31,37,44,49,50,50,80];
      | B=[-41.5,-41.5,-63,-20,-63,-20,-63,-20,-41.5,-41.5,-41.5,-34,-26,-21,-20,-22,-28,-37,-47,-57,-63,-63,-54,-44,-34,-26,-21,-20,-22,-28,-37,-47,-57,-63,-63,-54,-44,-34,-26,-21,-20,-22,-28,-37,-47,-57,-63,-63,-54,-44,-34,-26,-21,-20,-22,-28,-37,-41.50,-41.5];
      | plot(A,B);
      | color('black');
      | port_label('LConn', 1, '+')
  12 : Subsystem
  12 Y PQ : Subsystem  mask(Single Phase ZIP Load){Vnom=1.0*2401.78, fnom=60, Pnom=20e3*a, Qnom=10e3*a, LoadType=constant P, Vlim=0.7}
      mask prompts: Vnom "Nominal Voltage Vn (Vrms)"; fnom "Nominal Frequency fn (Hz)"; Pnom "Nominal Active power (W)"; Qnom "Nominal Reactive power (VAR)"; LoadType "Load Type"; Vlim "Minimum voltage (pu)"
      mask help:
      | Notes:
      | Single Phase ZIP load model which gets converted to constant Z type if the voltage becomes lower than the Minimum Voltage.
      mask TypeOptions LoadType: Constant Z | constant I | constant P
      mask DialogControl ParameterTabVar0 Prompt: Parameters
      mask DialogControl ParameterTabVar1 Prompt: Type
      mask Display:
      | color('red');
      | A=[-210,-180,-170,-160,-147,-140,-130,-120,-110,-80,-50,-49,-45,-39,-33,-26,-21,-18,-17,-19,-22,-22,-26,-27,-25,-22,-16,-9,-3,2,6,6,4,1,1,-3,-4,-2,2,7,14,20,26,29,30,28,24,24,21,20,21,25,31,37,44,49,50,50,80];
      | B=[-41.5,-41.5,-63,-20,-63,-20,-63,-20,-41.5,-41.5,-41.5,-34,-26,-21,-20,-22,-28,-37,-47,-57,-63,-63,-54,-44,-34,-26,-21,-20,-22,-28,-37,-47,-57,-63,-63,-54,-44,-34,-26,-21,-20,-22,-28,-37,-47,-57,-63,-63,-54,-44,-34,-26,-21,-20,-22,-28,-37,-41.50,-41.5];
      | plot(A,B);
      | color('black');
      | port_label('LConn', 1, '+')
  13 : powerlib/Measurements/Three-Phase V-I Measurement  VoltageMeasurement=phase-to-ground  SetLabelV=on  LabelV=V13  Vpu=off  VpuLL=off  CurrentMeasurement=no  SetLabelI=on  LabelI=I800  Ipu=off  Pbase=100e6  Vbase=24900  OutputType=Complex  PhasorSimulation=on  PSBequivalent=0
      settings: SourceProductName=Simscape Electrical
  13-152 : powerlib/Elements/Three-Phase Breaker  InitialState=closed  SwitchA=off  SwitchB=off  SwitchC=off  SwitchTimes="[1/60  5/60]"  External=off  BreakerResistance=1e-6  SnubberResistance=1e6  SnubberCapacitance=inf  Measurements=None
      settings: SourceProductName=Simscape Electrical
  13-18 2 : powerlib/Elements/Three-Phase PI Section Line  LConnTagsString=a|b|c  RConnTagsString=A|B|C  Frequency=60  Resistances=[R1_2 R0_2]  Inductances=[L1_2 L0_2]  Capacitances=[C1_2 C0_2]  Length=825*ft2km
      settings: SourceProductName=Simscape Electrical
  13-34 11 : powerlib/Elements/Pi Section Line  LConnTagsString=__new0  RConnTagsString=__new0  Frequency=60  Resistance=R1_11  Inductance=L1_11  Capacitance=C1_11  Length=150*ft2km  PiSections=1  Measurements=None
      settings: AttributesFormatString=\n  SourceProductName=Simscape Electrical  SourceProductBaseCode=PS
  135 : powerlib/Measurements/Three-Phase V-I Measurement  VoltageMeasurement=phase-to-ground  SetLabelV=on  LabelV=V135  Vpu=off  VpuLL=off  CurrentMeasurement=no  SetLabelI=on  LabelI=I800  Ipu=off  Pbase=100e6  Vbase=24900  OutputType=Complex  PhasorSimulation=on  PSBequivalent=0
      settings: SourceProductName=Simscape Electrical
  135-35 4 : powerlib/Elements/Three-Phase PI Section Line  LConnTagsString=a|b|c  RConnTagsString=A|B|C  Frequency=60  Resistances=[R1_4 R0_4]  Inductances=[L1_4 L0_4]  Capacitances=[C1_4 C0_4]  Length=375*ft2km
      settings: SourceProductName=Simscape Electrical
  14 : Subsystem
  14-10 9 : powerlib/Elements/Pi Section Line  LConnTagsString=__new0  RConnTagsString=__new0  Frequency=60  Resistance=R1_9  Inductance=L1_9  Capacitance=C1_9  Length=250*ft2km  PiSections=1  Measurements=None
      settings: AttributesFormatString=\n  SourceProductName=Simscape Electrical  SourceProductBaseCode=PS
  14-11 9 : powerlib/Elements/Pi Section Line  LConnTagsString=__new0  RConnTagsString=__new0  Frequency=60  Resistance=R1_9  Inductance=L1_9  Capacitance=C1_9  Length=250*ft2km  PiSections=1  Measurements=None
      settings: AttributesFormatString=\n  SourceProductName=Simscape Electrical  SourceProductBaseCode=PS
  149 : powerlib/Measurements/Three-Phase V-I Measurement  VoltageMeasurement=phase-to-ground  SetLabelV=on  LabelV=V149  Vpu=off  VpuLL=off  CurrentMeasurement=no  SetLabelI=on  LabelI=I800  Ipu=off  Pbase=100e6  Vbase=24900  OutputType=Complex  PhasorSimulation=on  PSBequivalent=0
      settings: SourceProductName=Simscape Electrical
  149-1 1 : Subsystem  mask(Three-Phase PI Section Block){Rl=R_1, Ll=L_1, Cl=C_1, L=400*ft2km}
      mask prompts: Rl "Resistance per unit Length(Ohm/Km)[3x3 matrix]"; Ll "Inductance per unit Length(H/Km)[3x3 matrix]"; Cl "Capacitance per unit Length(F/Km)[3x3 matrix]"; L "Length (Km)"
      mask help: This block models a three-phase transmission line with a single PI section.
  15 : Subsystem
  15-16 11 : powerlib/Elements/Pi Section Line  LConnTagsString=__new0  RConnTagsString=__new0  Frequency=60  Resistance=R1_11  Inductance=L1_11  Capacitance=C1_11  Length=375*ft2km  PiSections=1  Measurements=None
      settings: AttributesFormatString=\n  SourceProductName=Simscape Electrical  SourceProductBaseCode=PS
  15-17 11 : powerlib/Elements/Pi Section Line  LConnTagsString=__new0  RConnTagsString=__new0  Frequency=60  Resistance=R1_11  Inductance=L1_11  Capacitance=C1_11  Length=350*ft2km  PiSections=1  Measurements=None
      settings: AttributesFormatString=\n  SourceProductName=Simscape Electrical  SourceProductBaseCode=PS
  150 : powerlib/Measurements/Three-Phase V-I Measurement  VoltageMeasurement=phase-to-ground  SetLabelV=on  LabelV=V150  Vpu=off  VpuLL=off  CurrentMeasurement=yes  SetLabelI=on  LabelI=I150  Ipu=off  Pbase=100e6  Vbase=24900  OutputType=Complex  PhasorSimulation=on  PSBequivalent=0
      settings: SourceProductName=Simscape Electrical
  150-1 : powerlib/Elements/Three-Phase Breaker  InitialState=closed  SwitchA=off  SwitchB=off  SwitchC=off  SwitchTimes="[1/60  5/60]"  External=off  BreakerResistance=1e-6  SnubberResistance=1e6  SnubberCapacitance=inf  Measurements=None
      settings: SourceProductName=Simscape Electrical
  151 : powerlib/Measurements/Three-Phase V-I Measurement  VoltageMeasurement=phase-to-ground  SetLabelV=on  LabelV=V151  Vpu=off  VpuLL=off  CurrentMeasurement=no  SetLabelI=on  LabelI=I65  Ipu=off  Pbase=100e6  Vbase=24900  OutputType=Complex  PhasorSimulation=on  PSBequivalent=0
      settings: SourceProductName=Simscape Electrical
  151-1 : powerlib/Elements/Three-Phase Breaker  InitialState=open  SwitchA=off  SwitchB=off  SwitchC=off  SwitchTimes="[1/60  5/60]"  External=off  BreakerResistance=0.01  SnubberResistance=1e6  SnubberCapacitance=inf  Measurements=None
      settings: SourceProductName=Simscape Electrical
  152 : powerlib/Measurements/Three-Phase V-I Measurement  VoltageMeasurement=phase-to-ground  SetLabelV=on  LabelV=V152  Vpu=off  VpuLL=off  CurrentMeasurement=no  SetLabelI=on  LabelI=I65  Ipu=off  Pbase=100e6  Vbase=24900  OutputType=Complex  PhasorSimulation=on  PSBequivalent=0
      settings: SourceProductName=Simscape Electrical
  152-52 1 : powerlib/Elements/Three-Phase PI Section Line  LConnTagsString=a|b|c  RConnTagsString=A|B|C  Frequency=60  Resistances=[R1_1 R0_1]  Inductances=[L1_1 L0_1]  Capacitances=[C1_1 C0_1]  Length=400*ft2km
      settings: SourceProductName=Simscape Electrical
  16 : Subsystem
  16 Y PQ : Subsystem  mask(Single Phase ZIP Load){Vnom=1.0*2401.78, fnom=60, Pnom=40e3*a, Qnom=20e3*a, LoadType=constant P, Vlim=0.7}
      mask prompts: Vnom "Nominal Voltage Vn (Vrms)"; fnom "Nominal Frequency fn (Hz)"; Pnom "Nominal Active power (W)"; Qnom "Nominal Reactive power (VAR)"; LoadType "Load Type"; Vlim "Minimum voltage (pu)"
      mask help:
      | Notes:
      | Single Phase ZIP load model which gets converted to constant Z type if the voltage becomes lower than the Minimum Voltage.
      mask TypeOptions LoadType: Constant Z | constant I | constant P
      mask DialogControl ParameterTabVar0 Prompt: Parameters
      mask DialogControl ParameterTabVar1 Prompt: Type
      mask Display:
      | color('red');
      | A=[-210,-180,-170,-160,-147,-140,-130,-120,-110,-80,-50,-49,-45,-39,-33,-26,-21,-18,-17,-19,-22,-22,-26,-27,-25,-22,-16,-9,-3,2,6,6,4,1,1,-3,-4,-2,2,7,14,20,26,29,30,28,24,24,21,20,21,25,31,37,44,49,50,50,80];
      | B=[-41.5,-41.5,-63,-20,-63,-20,-63,-20,-41.5,-41.5,-41.5,-34,-26,-21,-20,-22,-28,-37,-47,-57,-63,-63,-54,-44,-34,-26,-21,-20,-22,-28,-37,-47,-57,-63,-63,-54,-44,-34,-26,-21,-20,-22,-28,-37,-47,-57,-63,-63,-54,-44,-34,-26,-21,-20,-22,-28,-37,-41.50,-41.5];
      | plot(A,B);
      | color('black');
      | port_label('LConn', 1, '+')
  160 : powerlib/Measurements/Three-Phase V-I Measurement  VoltageMeasurement=phase-to-ground  SetLabelV=on  LabelV=V160  Vpu=off  VpuLL=off  CurrentMeasurement=no  SetLabelI=on  LabelI=I65  Ipu=off  Pbase=100e6  Vbase=24900  OutputType=Complex  PhasorSimulation=on  PSBequivalent=0
      settings: SourceProductName=Simscape Electrical
  160-67 6 : Subsystem  mask(Three-Phase PI Section Block){Rl=R_6, Ll=L_6, Cl=C_6, L=350*ft2km}
      mask prompts: Rl "Resistance per unit Length(Ohm/Km)[3x3 matrix]"; Ll "Inductance per unit Length(H/Km)[3x3 matrix]"; Cl "Capacitance per unit Length(F/Km)[3x3 matrix]"; L "Length (Km)"
      mask help: This block models a three-phase transmission line with a single PI section.
  17 : Subsystem
  17 Y PQ : Subsystem  mask(Single Phase ZIP Load){Vnom=1.0*2401.78, fnom=60, Pnom=20e3*a, Qnom=10e3*a, LoadType=constant P, Vlim=0.7}
      mask prompts: Vnom "Nominal Voltage Vn (Vrms)"; fnom "Nominal Frequency fn (Hz)"; Pnom "Nominal Active power (W)"; Qnom "Nominal Reactive power (VAR)"; LoadType "Load Type"; Vlim "Minimum voltage (pu)"
      mask help:
      | Notes:
      | Single Phase ZIP load model which gets converted to constant Z type if the voltage becomes lower than the Minimum Voltage.
      mask TypeOptions LoadType: Constant Z | constant I | constant P
      mask DialogControl ParameterTabVar0 Prompt: Parameters
      mask DialogControl ParameterTabVar1 Prompt: Type
      mask Display:
      | color('red');
      | A=[-210,-180,-170,-160,-147,-140,-130,-120,-110,-80,-50,-49,-45,-39,-33,-26,-21,-18,-17,-19,-22,-22,-26,-27,-25,-22,-16,-9,-3,2,6,6,4,1,1,-3,-4,-2,2,7,14,20,26,29,30,28,24,24,21,20,21,25,31,37,44,49,50,50,80];
      | B=[-41.5,-41.5,-63,-20,-63,-20,-63,-20,-41.5,-41.5,-41.5,-34,-26,-21,-20,-22,-28,-37,-47,-57,-63,-63,-54,-44,-34,-26,-21,-20,-22,-28,-37,-47,-57,-63,-63,-54,-44,-34,-26,-21,-20,-22,-28,-37,-47,-57,-63,-63,-54,-44,-34,-26,-21,-20,-22,-28,-37,-41.50,-41.5];
      | plot(A,B);
      | color('black');
      | port_label('LConn', 1, '+')
  18 : powerlib/Measurements/Three-Phase V-I Measurement  VoltageMeasurement=phase-to-ground  SetLabelV=on  LabelV=V18  Vpu=off  VpuLL=off  CurrentMeasurement=no  SetLabelI=on  LabelI=I800  Ipu=off  Pbase=100e6  Vbase=24900  OutputType=Complex  PhasorSimulation=on  PSBequivalent=0
      settings: SourceProductName=Simscape Electrical
  18-135 : powerlib/Elements/Three-Phase Breaker  InitialState=closed  SwitchA=off  SwitchB=off  SwitchC=off  SwitchTimes="[1/60  5/60]"  External=off  BreakerResistance=1e-6  SnubberResistance=1e6  SnubberCapacitance=inf  Measurements=None
      settings: SourceProductName=Simscape Electrical
  18-19 9 : powerlib/Elements/Pi Section Line  LConnTagsString=__new0  RConnTagsString=__new0  Frequency=60  Resistance=R1_9  Inductance=L1_9  Capacitance=C1_9  Length=250*ft2km  PiSections=1  Measurements=None
      settings: AttributesFormatString=\n  SourceProductName=Simscape Electrical  SourceProductBaseCode=PS
  18-21 2 : powerlib/Elements/Three-Phase PI Section Line  LConnTagsString=a|b|c  RConnTagsString=A|B|C  Frequency=60  Resistances=[R1_2 R0_2]  Inductances=[L1_2 L0_2]  Capacitances=[C1_2 C0_2]  Length=300*ft2km
      settings: SourceProductName=Simscape Electrical
  19 : Subsystem
  19 Y PQ : Subsystem  mask(Single Phase ZIP Load){Vnom=1.0*2401.78, fnom=60, Pnom=40e3*a, Qnom=20e3*a, LoadType=constant P, Vlim=0.7}
      mask prompts: Vnom "Nominal Voltage Vn (Vrms)"; fnom "Nominal Frequency fn (Hz)"; Pnom "Nominal Active power (W)"; Qnom "Nominal Reactive power (VAR)"; LoadType "Load Type"; Vlim "Minimum voltage (pu)"
      mask help:
      | Notes:
      | Single Phase ZIP load model which gets converted to constant Z type if the voltage becomes lower than the Minimum Voltage.
      mask TypeOptions LoadType: Constant Z | constant I | constant P
      mask DialogControl ParameterTabVar0 Prompt: Parameters
      mask DialogControl ParameterTabVar1 Prompt: Type
      mask Display:
      | color('red');
      | A=[-210,-180,-170,-160,-147,-140,-130,-120,-110,-80,-50,-49,-45,-39,-33,-26,-21,-18,-17,-19,-22,-22,-26,-27,-25,-22,-16,-9,-3,2,6,6,4,1,1,-3,-4,-2,2,7,14,20,26,29,30,28,24,24,21,20,21,25,31,37,44,49,50,50,80];
      | B=[-41.5,-41.5,-63,-20,-63,-20,-63,-20,-41.5,-41.5,-41.5,-34,-26,-21,-20,-22,-28,-37,-47,-57,-63,-63,-54,-44,-34,-26,-21,-20,-22,-28,-37,-47,-57,-63,-63,-54,-44,-34,-26,-21,-20,-22,-28,-37,-47,-57,-63,-63,-54,-44,-34,-26,-21,-20,-22,-28,-37,-41.50,-41.5];
      | plot(A,B);
      | color('black');
      | port_label('LConn', 1, '+')
  19-20 9 : powerlib/Elements/Pi Section Line  LConnTagsString=__new0  RConnTagsString=__new0  Frequency=60  Resistance=R1_9  Inductance=L1_9  Capacitance=C1_9  Length=325*ft2km  PiSections=1  Measurements=None
      settings: AttributesFormatString=\n  SourceProductName=Simscape Electrical  SourceProductBaseCode=PS
  197 : powerlib/Measurements/Three-Phase V-I Measurement  VoltageMeasurement=phase-to-ground  SetLabelV=on  LabelV=V197  Vpu=off  VpuLL=off  CurrentMeasurement=no  SetLabelI=on  LabelI=I65  Ipu=off  Pbase=100e6  Vbase=24900  OutputType=Complex  PhasorSimulation=on  PSBequivalent=0
      settings: SourceProductName=Simscape Electrical
  197-101 3 : powerlib/Elements/Three-Phase PI Section Line  LConnTagsString=a|b|c  RConnTagsString=A|B|C  Frequency=60  Resistances=[R1_3 R0_3]  Inductances=[L1_3 L0_3]  Capacitances=[C1_3 C0_3]  Length=250*ft2km
      settings: SourceProductName=Simscape Electrical
  2 : Subsystem
  2 Y PQ : Subsystem  mask(Single Phase ZIP Load){Vnom=1.0*2401.78, fnom=60, Pnom=20e3*a, Qnom=10e3*a, LoadType=constant P, Vlim=0.7}
      mask prompts: Vnom "Nominal Voltage Vn (Vrms)"; fnom "Nominal Frequency fn (Hz)"; Pnom "Nominal Active power (W)"; Qnom "Nominal Reactive power (VAR)"; LoadType "Load Type"; Vlim "Minimum voltage (pu)"
      mask help:
      | Notes:
      | Single Phase ZIP load model which gets converted to constant Z type if the voltage becomes lower than the Minimum Voltage.
      mask TypeOptions LoadType: Constant Z | constant I | constant P
      mask DialogControl ParameterTabVar0 Prompt: Parameters
      mask DialogControl ParameterTabVar1 Prompt: Type
      mask Display:
      | color('red');
      | A=[-210,-180,-170,-160,-147,-140,-130,-120,-110,-80,-50,-49,-45,-39,-33,-26,-21,-18,-17,-19,-22,-22,-26,-27,-25,-22,-16,-9,-3,2,6,6,4,1,1,-3,-4,-2,2,7,14,20,26,29,30,28,24,24,21,20,21,25,31,37,44,49,50,50,80];
      | B=[-41.5,-41.5,-63,-20,-63,-20,-63,-20,-41.5,-41.5,-41.5,-34,-26,-21,-20,-22,-28,-37,-47,-57,-63,-63,-54,-44,-34,-26,-21,-20,-22,-28,-37,-47,-57,-63,-63,-54,-44,-34,-26,-21,-20,-22,-28,-37,-47,-57,-63,-63,-54,-44,-34,-26,-21,-20,-22,-28,-37,-41.50,-41.5];
      | plot(A,B);
      | color('black');
      | port_label('LConn', 1, '+')
  20 : Subsystem
  20 Y I : Subsystem  mask(Single Phase ZIP Load){Vnom=1.0*2401.78, fnom=60, Pnom=40e3*a, Qnom=20e3*a, LoadType=constant I, Vlim=0.7}
      mask prompts: Vnom "Nominal Voltage Vn (Vrms)"; fnom "Nominal Frequency fn (Hz)"; Pnom "Nominal Active power (W)"; Qnom "Nominal Reactive power (VAR)"; LoadType "Load Type"; Vlim "Minimum voltage (pu)"
      mask help:
      | Notes:
      | Single Phase ZIP load model which gets converted to constant Z type if the voltage becomes lower than the Minimum Voltage.
      mask TypeOptions LoadType: Constant Z | constant I | constant P
      mask DialogControl ParameterTabVar0 Prompt: Parameters
      mask DialogControl ParameterTabVar1 Prompt: Type
      mask Display:
      | color('red');
      | A=[-210,-180,-170,-160,-147,-140,-130,-120,-110,-80,-50,-49,-45,-39,-33,-26,-21,-18,-17,-19,-22,-22,-26,-27,-25,-22,-16,-9,-3,2,6,6,4,1,1,-3,-4,-2,2,7,14,20,26,29,30,28,24,24,21,20,21,25,31,37,44,49,50,50,80];
      | B=[-41.5,-41.5,-63,-20,-63,-20,-63,-20,-41.5,-41.5,-41.5,-34,-26,-21,-20,-22,-28,-37,-47,-57,-63,-63,-54,-44,-34,-26,-21,-20,-22,-28,-37,-47,-57,-63,-63,-54,-44,-34,-26,-21,-20,-22,-28,-37,-47,-57,-63,-63,-54,-44,-34,-26,-21,-20,-22,-28,-37,-41.50,-41.5];
      | plot(A,B);
      | color('black');
      | port_label('LConn', 1, '+')
  21 : powerlib/Measurements/Three-Phase V-I Measurement  VoltageMeasurement=phase-to-ground  SetLabelV=on  LabelV=V21  Vpu=off  VpuLL=off  CurrentMeasurement=no  SetLabelI=on  LabelI=I800  Ipu=off  Pbase=100e6  Vbase=24900  OutputType=Complex  PhasorSimulation=on  PSBequivalent=0
      settings: SourceProductName=Simscape Electrical
  21-22 10 : powerlib/Elements/Pi Section Line  LConnTagsString=__new0  RConnTagsString=__new0  Frequency=60  Resistance=R1_10  Inductance=L1_10  Capacitance=C1_10  Length=525*ft2km  PiSections=1  Measurements=None
      settings: AttributesFormatString=\n  SourceProductName=Simscape Electrical  SourceProductBaseCode=PS
  21-23 2 : powerlib/Elements/Three-Phase PI Section Line  LConnTagsString=a|b|c  RConnTagsString=A|B|C  Frequency=60  Resistances=[R1_2 R0_2]  Inductances=[L1_2 L0_2]  Capacitances=[C1_2 C0_2]  Length=250*ft2km
      settings: SourceProductName=Simscape Electrical
  22 : Subsystem
  22 Y Z : Subsystem  mask(Single Phase ZIP Load){Vnom=1.0*2401.78, fnom=60, Pnom=40e3*a, Qnom=20e3*a, LoadType=Constant Z, Vlim=0.7}
      mask prompts: Vnom "Nominal Voltage Vn (Vrms)"; fnom "Nominal Frequency fn (Hz)"; Pnom "Nominal Active power (W)"; Qnom "Nominal Reactive power (VAR)"; LoadType "Load Type"; Vlim "Minimum voltage (pu)"
      mask help:
      | Notes:
      | Single Phase ZIP load model which gets converted to constant Z type if the voltage becomes lower than the Minimum Voltage.
      mask TypeOptions LoadType: Constant Z | constant I | constant P
      mask DialogControl ParameterTabVar0 Prompt: Parameters
      mask DialogControl ParameterTabVar1 Prompt: Type
      mask Display:
      | color('red');
      | A=[-210,-180,-170,-160,-147,-140,-130,-120,-110,-80,-50,-49,-45,-39,-33,-26,-21,-18,-17,-19,-22,-22,-26,-27,-25,-22,-16,-9,-3,2,6,6,4,1,1,-3,-4,-2,2,7,14,20,26,29,30,28,24,24,21,20,21,25,31,37,44,49,50,50,80];
      | B=[-41.5,-41.5,-63,-20,-63,-20,-63,-20,-41.5,-41.5,-41.5,-34,-26,-21,-20,-22,-28,-37,-47,-57,-63,-63,-54,-44,-34,-26,-21,-20,-22,-28,-37,-47,-57,-63,-63,-54,-44,-34,-26,-21,-20,-22,-28,-37,-47,-57,-63,-63,-54,-44,-34,-26,-21,-20,-22,-28,-37,-41.50,-41.5];
      | plot(A,B);
      | color('black');
      | port_label('LConn', 1, '+')
  23 : powerlib/Measurements/Three-Phase V-I Measurement  VoltageMeasurement=phase-to-ground  SetLabelV=on  LabelV=V23  Vpu=off  VpuLL=off  CurrentMeasurement=no  SetLabelI=on  LabelI=I800  Ipu=off  Pbase=100e6  Vbase=24900  OutputType=Complex  PhasorSimulation=on  PSBequivalent=0
      settings: SourceProductName=Simscape Electrical
  23-24 11 : powerlib/Elements/Pi Section Line  LConnTagsString=__new0  RConnTagsString=__new0  Frequency=60  Resistance=R1_11  Inductance=L1_11  Capacitance=C1_11  Length=550*ft2km  PiSections=1  Measurements=None
      settings: AttributesFormatString=\n  SourceProductName=Simscape Electrical  SourceProductBaseCode=PS
  23-25 2 : powerlib/Elements/Three-Phase PI Section Line  LConnTagsString=a|b|c  RConnTagsString=A|B|C  Frequency=60  Resistances=[R1_2 R0_2]  Inductances=[L1_2 L0_2]  Capacitances=[C1_2 C0_2]  Length=275*ft2km
      settings: SourceProductName=Simscape Electrical
  24 : Subsystem
  24 Y PQ : Subsystem  mask(Single Phase ZIP Load){Vnom=1.0*2401.78, fnom=60, Pnom=40e3*a, Qnom=20e3*a, LoadType=constant P, Vlim=0.7}
      mask prompts: Vnom "Nominal Voltage Vn (Vrms)"; fnom "Nominal Frequency fn (Hz)"; Pnom "Nominal Active power (W)"; Qnom "Nominal Reactive power (VAR)"; LoadType "Load Type"; Vlim "Minimum voltage (pu)"
      mask help:
      | Notes:
      | Single Phase ZIP load model which gets converted to constant Z type if the voltage becomes lower than the Minimum Voltage.
      mask TypeOptions LoadType: Constant Z | constant I | constant P
      mask DialogControl ParameterTabVar0 Prompt: Parameters
      mask DialogControl ParameterTabVar1 Prompt: Type
      mask Display:
      | color('red');
      | A=[-210,-180,-170,-160,-147,-140,-130,-120,-110,-80,-50,-49,-45,-39,-33,-26,-21,-18,-17,-19,-22,-22,-26,-27,-25,-22,-16,-9,-3,2,6,6,4,1,1,-3,-4,-2,2,7,14,20,26,29,30,28,24,24,21,20,21,25,31,37,44,49,50,50,80];
      | B=[-41.5,-41.5,-63,-20,-63,-20,-63,-20,-41.5,-41.5,-41.5,-34,-26,-21,-20,-22,-28,-37,-47,-57,-63,-63,-54,-44,-34,-26,-21,-20,-22,-28,-37,-47,-57,-63,-63,-54,-44,-34,-26,-21,-20,-22,-28,-37,-47,-57,-63,-63,-54,-44,-34,-26,-21,-20,-22,-28,-37,-41.50,-41.5];
      | plot(A,B);
      | color('black');
      | port_label('LConn', 1, '+')
  25 : powerlib/Measurements/Three-Phase V-I Measurement  VoltageMeasurement=phase-to-ground  SetLabelV=on  LabelV=V25  Vpu=off  VpuLL=off  CurrentMeasurement=no  SetLabelI=on  LabelI=I800  Ipu=off  Pbase=100e6  Vbase=24900  OutputType=Complex  PhasorSimulation=on  PSBequivalent=0
      settings: SourceProductName=Simscape Electrical
  25-26 7 : Subsystem  mask{Rl=R_7, Ll=L_7, Cl=C_7, L=350*ft2km}
      mask prompts: Rl "Resistance per unit Length(Ohm/Km)[3x3 matrix]"; Ll "Inductance per unit Length(H/Km)[3x3 matrix]"; Cl "Capacitance per unit Length(F/Km)[3x3 matrix"; L "Length (Km)"
      mask init:
      | W = sign(sum(abs(Rl)));
      | s = find(W==1);%Identify non zero rows and columns
      | 
      | Rt =Rl(s,s);
      | Rl= Rt;
      | Lt =Ll(s,s);
      | Ll= Lt;
      | Ct =Cl(s,s);
      | Cl= Ct;
  25-28 2 : powerlib/Elements/Three-Phase PI Section Line  LConnTagsString=a|b|c  RConnTagsString=A|B|C  Frequency=60  Resistances=[R1_2 R0_2]  Inductances=[L1_2 L0_2]  Capacitances=[C1_2 C0_2]  Length=200*ft2km
      settings: SourceProductName=Simscape Electrical
  250 : powerlib/Measurements/Three-Phase V-I Measurement  VoltageMeasurement=phase-to-ground  SetLabelV=on  LabelV=V250  Vpu=off  VpuLL=off  CurrentMeasurement=no  SetLabelI=on  LabelI=I800  Ipu=off  Pbase=100e6  Vbase=24900  OutputType=Complex  PhasorSimulation=on  PSBequivalent=0
      settings: SourceProductName=Simscape Electrical
  250-251 : powerlib/Elements/Three-Phase Breaker  InitialState=open  SwitchA=on  SwitchB=on  SwitchC=on  SwitchTimes="[1/60  5/60]"  External=off  BreakerResistance=0.01  SnubberResistance=1e6  SnubberCapacitance=inf  Measurements=None
      settings: SourceProductName=Simscape Electrical
  26 : Subsystem
  26-31 11 : powerlib/Elements/Pi Section Line  LConnTagsString=__new0  RConnTagsString=__new0  Frequency=60  Resistance=R1_11  Inductance=L1_11  Capacitance=C1_11  Length=225*ft2km  PiSections=1  Measurements=None
      settings: AttributesFormatString=\n  SourceProductName=Simscape Electrical  SourceProductBaseCode=PS
  26-7 7 : Subsystem  mask{Rl=R_7, Ll=L_7, Cl=C_7, L=275*ft2km}
      mask prompts: Rl "Resistance per unit Length(Ohm/Km)[3x3 matrix]"; Ll "Inductance per unit Length(H/Km)[3x3 matrix]"; Cl "Capacitance per unit Length(F/Km)[3x3 matrix"; L "Length (Km)"
      mask init:
      | W = sign(sum(abs(Rl)));
      | s = find(W==1);%Identify non zero rows and columns
      | 
      | Rt =Rl(s,s);
      | Rl= Rt;
      | Lt =Ll(s,s);
      | Ll= Lt;
      | Ct =Cl(s,s);
      | Cl= Ct;
  27 : Subsystem
  27-33 9 : powerlib/Elements/Pi Section Line  LConnTagsString=__new0  RConnTagsString=__new0  Frequency=60  Resistance=R1_9  Inductance=L1_9  Capacitance=C1_9  Length=500*ft2km  PiSections=1  Measurements=None
      settings: AttributesFormatString=\n  SourceProductName=Simscape Electrical  SourceProductBaseCode=PS
  28 : powerlib/Measurements/Three-Phase V-I Measurement  VoltageMeasurement=phase-to-ground  SetLabelV=on  LabelV=V28  Vpu=off  VpuLL=off  CurrentMeasurement=no  SetLabelI=on  LabelI=I800  Ipu=off  Pbase=100e6  Vbase=24900  OutputType=Complex  PhasorSimulation=on  PSBequivalent=0
      settings: SourceProductName=Simscape Electrical
  28 Y I : Subsystem  mask(Single Phase ZIP Load){Vnom=1.0*2401.78, fnom=60, Pnom=40e3*a, Qnom=20e3*a, LoadType=constant I, Vlim=0.7}
      mask prompts: Vnom "Nominal Voltage Vn (Vrms)"; fnom "Nominal Frequency fn (Hz)"; Pnom "Nominal Active power (W)"; Qnom "Nominal Reactive power (VAR)"; LoadType "Load Type"; Vlim "Minimum voltage (pu)"
      mask help:
      | Notes:
      | Single Phase ZIP load model which gets converted to constant Z type if the voltage becomes lower than the Minimum Voltage.
      mask TypeOptions LoadType: Constant Z | constant I | constant P
      mask DialogControl ParameterTabVar0 Prompt: Parameters
      mask DialogControl ParameterTabVar1 Prompt: Type
      mask Display:
      | color('red');
      | A=[-210,-180,-170,-160,-147,-140,-130,-120,-110,-80,-50,-49,-45,-39,-33,-26,-21,-18,-17,-19,-22,-22,-26,-27,-25,-22,-16,-9,-3,2,6,6,4,1,1,-3,-4,-2,2,7,14,20,26,29,30,28,24,24,21,20,21,25,31,37,44,49,50,50,80];
      | B=[-41.5,-41.5,-63,-20,-63,-20,-63,-20,-41.5,-41.5,-41.5,-34,-26,-21,-20,-22,-28,-37,-47,-57,-63,-63,-54,-44,-34,-26,-21,-20,-22,-28,-37,-47,-57,-63,-63,-54,-44,-34,-26,-21,-20,-22,-28,-37,-47,-57,-63,-63,-54,-44,-34,-26,-21,-20,-22,-28,-37,-41.50,-41.5];
      | plot(A,B);
      | color('black');
      | port_label('LConn', 1, '+')
  28-29 2 : powerlib/Elements/Three-Phase PI Section Line  LConnTagsString=a|b|c  RConnTagsString=A|B|C  Frequency=60  Resistances=[R1_2 R0_2]  Inductances=[L1_2 L0_2]  Capacitances=[C1_2 C0_2]  Length=300*ft2km
      settings: SourceProductName=Simscape Electrical
  29 : powerlib/Measurements/Three-Phase V-I Measurement  VoltageMeasurement=phase-to-ground  SetLabelV=on  LabelV=V29  Vpu=off  VpuLL=off  CurrentMeasurement=no  SetLabelI=on  LabelI=I800  Ipu=off  Pbase=100e6  Vbase=24900  OutputType=Complex  PhasorSimulation=on  PSBequivalent=0
      settings: SourceProductName=Simscape Electrical
  29 Y Z : Subsystem  mask(Single Phase ZIP Load){Vnom=1.0*2401.78, fnom=60, Pnom=40e3*a, Qnom=20e3*a, LoadType=Constant Z, Vlim=0.7}
      mask prompts: Vnom "Nominal Voltage Vn (Vrms)"; fnom "Nominal Frequency fn (Hz)"; Pnom "Nominal Active power (W)"; Qnom "Nominal Reactive power (VAR)"; LoadType "Load Type"; Vlim "Minimum voltage (pu)"
      mask help:
      | Notes:
      | Single Phase ZIP load model which gets converted to constant Z type if the voltage becomes lower than the Minimum Voltage.
      mask TypeOptions LoadType: Constant Z | constant I | constant P
      mask DialogControl ParameterTabVar0 Prompt: Parameters
      mask DialogControl ParameterTabVar1 Prompt: Type
      mask Display:
      | color('red');
      | A=[-210,-180,-170,-160,-147,-140,-130,-120,-110,-80,-50,-49,-45,-39,-33,-26,-21,-18,-17,-19,-22,-22,-26,-27,-25,-22,-16,-9,-3,2,6,6,4,1,1,-3,-4,-2,2,7,14,20,26,29,30,28,24,24,21,20,21,25,31,37,44,49,50,50,80];
      | B=[-41.5,-41.5,-63,-20,-63,-20,-63,-20,-41.5,-41.5,-41.5,-34,-26,-21,-20,-22,-28,-37,-47,-57,-63,-63,-54,-44,-34,-26,-21,-20,-22,-28,-37,-47,-57,-63,-63,-54,-44,-34,-26,-21,-20,-22,-28,-37,-47,-57,-63,-63,-54,-44,-34,-26,-21,-20,-22,-28,-37,-41.50,-41.5];
      | plot(A,B);
      | color('black');
      | port_label('LConn', 1, '+')
  29-30 2 : powerlib/Elements/Three-Phase PI Section Line  LConnTagsString=a|b|c  RConnTagsString=A|B|C  Frequency=60  Resistances=[R1_2 R0_2]  Inductances=[L1_2 L0_2]  Capacitances=[C1_2 C0_2]  Length=350*ft2km
      settings: SourceProductName=Simscape Electrical
  3 : Subsystem
  3-4 11 : powerlib/Elements/Pi Section Line  LConnTagsString=__new0  RConnTagsString=__new0  Frequency=60  Resistance=R1_11  Inductance=L1_11  Capacitance=C1_11  Length=200*ft2km  PiSections=1  Measurements=None
      settings: AttributesFormatString=\n  SourceProductName=Simscape Electrical  SourceProductBaseCode=PS
  3-5 11 : powerlib/Elements/Pi Section Line  LConnTagsString=__new0  RConnTagsString=__new0  Frequency=60  Resistance=R1_11  Inductance=L1_11  Capacitance=C1_11  Length=325*ft2km  PiSections=1  Measurements=None
      settings: AttributesFormatString=\n  SourceProductName=Simscape Electrical  SourceProductBaseCode=PS
  "30 " : powerlib/Measurements/Three-Phase V-I Measurement  VoltageMeasurement=phase-to-ground  SetLabelV=on  LabelV=V30  Vpu=off  VpuLL=off  CurrentMeasurement=no  SetLabelI=on  LabelI=I800  Ipu=off  Pbase=100e6  Vbase=24900  OutputType=Complex  PhasorSimulation=on  PSBequivalent=0
      settings: SourceProductName=Simscape Electrical
  30 Y PQ : Subsystem  mask(Single Phase ZIP Load){Vnom=1.0*2401.78, fnom=60, Pnom=40e3*a, Qnom=20e3*a, LoadType=constant P, Vlim=0.7}
      mask prompts: Vnom "Nominal Voltage Vn (Vrms)"; fnom "Nominal Frequency fn (Hz)"; Pnom "Nominal Active power (W)"; Qnom "Nominal Reactive power (VAR)"; LoadType "Load Type"; Vlim "Minimum voltage (pu)"
      mask help:
      | Notes:
      | Single Phase ZIP load model which gets converted to constant Z type if the voltage becomes lower than the Minimum Voltage.
      mask TypeOptions LoadType: Constant Z | constant I | constant P
      mask DialogControl ParameterTabVar0 Prompt: Parameters
      mask DialogControl ParameterTabVar1 Prompt: Type
      mask Display:
      | color('red');
      | A=[-210,-180,-170,-160,-147,-140,-130,-120,-110,-80,-50,-49,-45,-39,-33,-26,-21,-18,-17,-19,-22,-22,-26,-27,-25,-22,-16,-9,-3,2,6,6,4,1,1,-3,-4,-2,2,7,14,20,26,29,30,28,24,24,21,20,21,25,31,37,44,49,50,50,80];
      | B=[-41.5,-41.5,-63,-20,-63,-20,-63,-20,-41.5,-41.5,-41.5,-34,-26,-21,-20,-22,-28,-37,-47,-57,-63,-63,-54,-44,-34,-26,-21,-20,-22,-28,-37,-47,-57,-63,-63,-54,-44,-34,-26,-21,-20,-22,-28,-37,-47,-57,-63,-63,-54,-44,-34,-26,-21,-20,-22,-28,-37,-41.50,-41.5];
      | plot(A,B);
      | color('black');
      | port_label('LConn', 1, '+')
  30-250 2 : powerlib/Elements/Three-Phase PI Section Line  LConnTagsString=a|b|c  RConnTagsString=A|B|C  Frequency=60  Resistances=[R1_2 R0_2]  Inductances=[L1_2 L0_2]  Capacitances=[C1_2 C0_2]  Length=200*ft2km
      settings: SourceProductName=Simscape Electrical
  300 : powerlib/Measurements/Three-Phase V-I Measurement  VoltageMeasurement=phase-to-ground  SetLabelV=on  LabelV=V300  Vpu=off  VpuLL=off  CurrentMeasurement=no  SetLabelI=on  LabelI=I65  Ipu=off  Pbase=100e6  Vbase=24900  OutputType=Complex  PhasorSimulation=on  PSBequivalent=0
      settings: SourceProductName=Simscape Electrical
  300-1 : powerlib/Elements/Three-Phase Breaker  InitialState=open  SwitchA=off  SwitchB=off  SwitchC=off  SwitchTimes="[1/60  5/60]"  External=off  BreakerResistance=0.01  SnubberResistance=1e6  SnubberCapacitance=inf  Measurements=None
      settings: SourceProductName=Simscape Electrical
  31 : Subsystem
  31 Y PQ : Subsystem  mask(Single Phase ZIP Load){Vnom=1.0*2401.78, fnom=60, Pnom=20e3*a, Qnom=10e3*a, LoadType=constant P, Vlim=0.7}
      mask prompts: Vnom "Nominal Voltage Vn (Vrms)"; fnom "Nominal Frequency fn (Hz)"; Pnom "Nominal Active power (W)"; Qnom "Nominal Reactive power (VAR)"; LoadType "Load Type"; Vlim "Minimum voltage (pu)"
      mask help:
      | Notes:
      | Single Phase ZIP load model which gets converted to constant Z type if the voltage becomes lower than the Minimum Voltage.
      mask TypeOptions LoadType: Constant Z | constant I | constant P
      mask DialogControl ParameterTabVar0 Prompt: Parameters
      mask DialogControl ParameterTabVar1 Prompt: Type
      mask Display:
      | color('red');
      | A=[-210,-180,-170,-160,-147,-140,-130,-120,-110,-80,-50,-49,-45,-39,-33,-26,-21,-18,-17,-19,-22,-22,-26,-27,-25,-22,-16,-9,-3,2,6,6,4,1,1,-3,-4,-2,2,7,14,20,26,29,30,28,24,24,21,20,21,25,31,37,44,49,50,50,80];
      | B=[-41.5,-41.5,-63,-20,-63,-20,-63,-20,-41.5,-41.5,-41.5,-34,-26,-21,-20,-22,-28,-37,-47,-57,-63,-63,-54,-44,-34,-26,-21,-20,-22,-28,-37,-47,-57,-63,-63,-54,-44,-34,-26,-21,-20,-22,-28,-37,-47,-57,-63,-63,-54,-44,-34,-26,-21,-20,-22,-28,-37,-41.50,-41.5];
      | plot(A,B);
      | color('black');
      | port_label('LConn', 1, '+')
  31-32 11 : powerlib/Elements/Pi Section Line  LConnTagsString=__new0  RConnTagsString=__new0  Frequency=60  Resistance=R1_11  Inductance=L1_11  Capacitance=C1_11  Length=300*ft2km  PiSections=1  Measurements=None
      settings: AttributesFormatString=\n  SourceProductName=Simscape Electrical  SourceProductBaseCode=PS
  32 : Subsystem
  32 Y PQ : Subsystem  mask(Single Phase ZIP Load){Vnom=1.0*2401.78, fnom=60, Pnom=20e3*a, Qnom=10e3*a, LoadType=constant P, Vlim=0.7}
      mask prompts: Vnom "Nominal Voltage Vn (Vrms)"; fnom "Nominal Frequency fn (Hz)"; Pnom "Nominal Active power (W)"; Qnom "Nominal Reactive power (VAR)"; LoadType "Load Type"; Vlim "Minimum voltage (pu)"
      mask help:
      | Notes:
      | Single Phase ZIP load model which gets converted to constant Z type if the voltage becomes lower than the Minimum Voltage.
      mask TypeOptions LoadType: Constant Z | constant I | constant P
      mask DialogControl ParameterTabVar0 Prompt: Parameters
      mask DialogControl ParameterTabVar1 Prompt: Type
      mask Display:
      | color('red');
      | A=[-210,-180,-170,-160,-147,-140,-130,-120,-110,-80,-50,-49,-45,-39,-33,-26,-21,-18,-17,-19,-22,-22,-26,-27,-25,-22,-16,-9,-3,2,6,6,4,1,1,-3,-4,-2,2,7,14,20,26,29,30,28,24,24,21,20,21,25,31,37,44,49,50,50,80];
      | B=[-41.5,-41.5,-63,-20,-63,-20,-63,-20,-41.5,-41.5,-41.5,-34,-26,-21,-20,-22,-28,-37,-47,-57,-63,-63,-54,-44,-34,-26,-21,-20,-22,-28,-37,-47,-57,-63,-63,-54,-44,-34,-26,-21,-20,-22,-28,-37,-47,-57,-63,-63,-54,-44,-34,-26,-21,-20,-22,-28,-37,-41.50,-41.5];
      | plot(A,B);
      | color('black');
      | port_label('LConn', 1, '+')
  33 : Subsystem
  33 Y I : Subsystem  mask(Single Phase ZIP Load){Vnom=1.0*2401.78, fnom=60, Pnom=40e3*a, Qnom=20e3*a, LoadType=constant I, Vlim=0.7}
      mask prompts: Vnom "Nominal Voltage Vn (Vrms)"; fnom "Nominal Frequency fn (Hz)"; Pnom "Nominal Active power (W)"; Qnom "Nominal Reactive power (VAR)"; LoadType "Load Type"; Vlim "Minimum voltage (pu)"
      mask help:
      | Notes:
      | Single Phase ZIP load model which gets converted to constant Z type if the voltage becomes lower than the Minimum Voltage.
      mask TypeOptions LoadType: Constant Z | constant I | constant P
      mask DialogControl ParameterTabVar0 Prompt: Parameters
      mask DialogControl ParameterTabVar1 Prompt: Type
      mask Display:
      | color('red');
      | A=[-210,-180,-170,-160,-147,-140,-130,-120,-110,-80,-50,-49,-45,-39,-33,-26,-21,-18,-17,-19,-22,-22,-26,-27,-25,-22,-16,-9,-3,2,6,6,4,1,1,-3,-4,-2,2,7,14,20,26,29,30,28,24,24,21,20,21,25,31,37,44,49,50,50,80];
      | B=[-41.5,-41.5,-63,-20,-63,-20,-63,-20,-41.5,-41.5,-41.5,-34,-26,-21,-20,-22,-28,-37,-47,-57,-63,-63,-54,-44,-34,-26,-21,-20,-22,-28,-37,-47,-57,-63,-63,-54,-44,-34,-26,-21,-20,-22,-28,-37,-47,-57,-63,-63,-54,-44,-34,-26,-21,-20,-22,-28,-37,-41.50,-41.5];
      | plot(A,B);
      | color('black');
      | port_label('LConn', 1, '+')
  34 : Subsystem
  34 Y Z : Subsystem  mask(Single Phase ZIP Load){Vnom=1.0*2401.78, fnom=60, Pnom=40e3*a, Qnom=20e3*a, LoadType=Constant Z, Vlim=0.7}
      mask prompts: Vnom "Nominal Voltage Vn (Vrms)"; fnom "Nominal Frequency fn (Hz)"; Pnom "Nominal Active power (W)"; Qnom "Nominal Reactive power (VAR)"; LoadType "Load Type"; Vlim "Minimum voltage (pu)"
      mask help:
      | Notes:
      | Single Phase ZIP load model which gets converted to constant Z type if the voltage becomes lower than the Minimum Voltage.
      mask TypeOptions LoadType: Constant Z | constant I | constant P
      mask DialogControl ParameterTabVar0 Prompt: Parameters
      mask DialogControl ParameterTabVar1 Prompt: Type
      mask Display:
      | color('red');
      | A=[-210,-180,-170,-160,-147,-140,-130,-120,-110,-80,-50,-49,-45,-39,-33,-26,-21,-18,-17,-19,-22,-22,-26,-27,-25,-22,-16,-9,-3,2,6,6,4,1,1,-3,-4,-2,2,7,14,20,26,29,30,28,24,24,21,20,21,25,31,37,44,49,50,50,80];
      | B=[-41.5,-41.5,-63,-20,-63,-20,-63,-20,-41.5,-41.5,-41.5,-34,-26,-21,-20,-22,-28,-37,-47,-57,-63,-63,-54,-44,-34,-26,-21,-20,-22,-28,-37,-47,-57,-63,-63,-54,-44,-34,-26,-21,-20,-22,-28,-37,-47,-57,-63,-63,-54,-44,-34,-26,-21,-20,-22,-28,-37,-41.50,-41.5];
      | plot(A,B);
      | color('black');
      | port_label('LConn', 1, '+')
  34-15 11 : powerlib/Elements/Pi Section Line  LConnTagsString=__new0  RConnTagsString=__new0  Frequency=60  Resistance=R1_11  Inductance=L1_11  Capacitance=C1_11  Length=100*ft2km  PiSections=1  Measurements=None
      settings: AttributesFormatString=\n  SourceProductName=Simscape Electrical  SourceProductBaseCode=PS
  35 : powerlib/Measurements/Three-Phase V-I Measurement  VoltageMeasurement=phase-to-ground  SetLabelV=on  LabelV=V35  Vpu=off  VpuLL=off  CurrentMeasurement=no  SetLabelI=on  LabelI=I800  Ipu=off  Pbase=100e6  Vbase=24900  OutputType=Complex  PhasorSimulation=on  PSBequivalent=0
      settings: SourceProductName=Simscape Electrical
  35 D PQ : Subsystem  mask(Single Phase ZIP Load){Vnom=1.0*2401.78, fnom=60, Pnom=40e3*a, Qnom=20e3*a, LoadType=constant P, Vlim=0.7}
      mask prompts: Vnom "Nominal Voltage Vn (Vrms)"; fnom "Nominal Frequency fn (Hz)"; Pnom "Nominal Active power (W)"; Qnom "Nominal Reactive power (VAR)"; LoadType "Load Type"; Vlim "Minimum voltage (pu)"
      mask help:
      | Notes:
      | Single Phase ZIP load model which gets converted to constant Z type if the voltage becomes lower than the Minimum Voltage.
      mask TypeOptions LoadType: Constant Z | constant I | constant P
      mask DialogControl ParameterTabVar0 Prompt: Parameters
      mask DialogControl ParameterTabVar1 Prompt: Type
      mask Display:
      | color('red');
      | A=[-210,-180,-170,-160,-147,-140,-130,-120,-110,-80,-50,-49,-45,-39,-33,-26,-21,-18,-17,-19,-22,-22,-26,-27,-25,-22,-16,-9,-3,2,6,6,4,1,1,-3,-4,-2,2,7,14,20,26,29,30,28,24,24,21,20,21,25,31,37,44,49,50,50,80];
      | B=[-41.5,-41.5,-63,-20,-63,-20,-63,-20,-41.5,-41.5,-41.5,-34,-26,-21,-20,-22,-28,-37,-47,-57,-63,-63,-54,-44,-34,-26,-21,-20,-22,-28,-37,-47,-57,-63,-63,-54,-44,-34,-26,-21,-20,-22,-28,-37,-47,-57,-63,-63,-54,-44,-34,-26,-21,-20,-22,-28,-37,-41.50,-41.5];
      | plot(A,B);
      | color('black');
      | port_label('LConn', 1, '+')
  35-36 8 : Subsystem  mask(Three-Phase PI Section Block){Rl=R_8, Ll=L_8, Cl=C_8, L=650*ft2km}
      mask prompts: Rl "Resistance per unit Length(Ohm/Km)[3x3 matrix]"; Ll "Inductance per unit Length(H/Km)[3x3 matrix]"; Cl "Capacitance per unit Length(F/Km)[3x3 matrix"; L "Length (Km)"
      mask help: This block models a two-phase transmission line with a single PI section.
      mask init:
      | W = sign(sum(abs(Rl)));
      | s = find(W==1);%Identify non zero rows and columns
      | 
      | Rt =Rl(s,s);
      | Rl= Rt;
      | Lt =Ll(s,s);
      | Ll= Lt;
      | Ct =Cl(s,s);
      | Cl= Ct;
  35-40 1 : powerlib/Elements/Three-Phase PI Section Line  LConnTagsString=a|b|c  RConnTagsString=A|B|C  Frequency=60  Resistances=[R1_1 R0_1]  Inductances=[L1_1 L0_1]  Capacitances=[C1_1 C0_1]  Length=250*ft2km
      settings: SourceProductName=Simscape Electrical
  36 : Subsystem
  36-37 9 : powerlib/Elements/Pi Section Line  LConnTagsString=__new0  RConnTagsString=__new0  Frequency=60  Resistance=R1_9  Inductance=L1_9  Capacitance=C1_9  Length=300*ft2km  PiSections=1  Measurements=None
      settings: AttributesFormatString=\n  SourceProductName=Simscape Electrical  SourceProductBaseCode=PS
  36-38 10 : powerlib/Elements/Pi Section Line  LConnTagsString=__new0  RConnTagsString=__new0  Frequency=60  Resistance=R1_10  Inductance=L1_10  Capacitance=C1_10  Length=250*ft2km  PiSections=1  Measurements=None
      settings: AttributesFormatString=\n  SourceProductName=Simscape Electrical  SourceProductBaseCode=PS
  37 : Subsystem
  37 Y Z : Subsystem  mask(Single Phase ZIP Load){Vnom=1.0*2401.78, fnom=60, Pnom=40e3*a, Qnom=20e3*a, LoadType=Constant Z, Vlim=0.7}
      mask prompts: Vnom "Nominal Voltage Vn (Vrms)"; fnom "Nominal Frequency fn (Hz)"; Pnom "Nominal Active power (W)"; Qnom "Nominal Reactive power (VAR)"; LoadType "Load Type"; Vlim "Minimum voltage (pu)"
      mask help:
      | Notes:
      | Single Phase ZIP load model which gets converted to constant Z type if the voltage becomes lower than the Minimum Voltage.
      mask TypeOptions LoadType: Constant Z | constant I | constant P
      mask DialogControl ParameterTabVar0 Prompt: Parameters
      mask DialogControl ParameterTabVar1 Prompt: Type
      mask Display:
      | color('red');
      | A=[-210,-180,-170,-160,-147,-140,-130,-120,-110,-80,-50,-49,-45,-39,-33,-26,-21,-18,-17,-19,-22,-22,-26,-27,-25,-22,-16,-9,-3,2,6,6,4,1,1,-3,-4,-2,2,7,14,20,26,29,30,28,24,24,21,20,21,25,31,37,44,49,50,50,80];
      | B=[-41.5,-41.5,-63,-20,-63,-20,-63,-20,-41.5,-41.5,-41.5,-34,-26,-21,-20,-22,-28,-37,-47,-57,-63,-63,-54,-44,-34,-26,-21,-20,-22,-28,-37,-47,-57,-63,-63,-54,-44,-34,-26,-21,-20,-22,-28,-37,-47,-57,-63,-63,-54,-44,-34,-26,-21,-20,-22,-28,-37,-41.50,-41.5];
      | plot(A,B);
      | color('black');
      | port_label('LConn', 1, '+')
  38 : Subsystem
  38 Y I : Subsystem  mask(Single Phase ZIP Load){Vnom=1.0*2401.78, fnom=60, Pnom=20e3*a, Qnom=10e3*a, LoadType=constant I, Vlim=0.7}
      mask prompts: Vnom "Nominal Voltage Vn (Vrms)"; fnom "Nominal Frequency fn (Hz)"; Pnom "Nominal Active power (W)"; Qnom "Nominal Reactive power (VAR)"; LoadType "Load Type"; Vlim "Minimum voltage (pu)"
      mask help:
      | Notes:
      | Single Phase ZIP load model which gets converted to constant Z type if the voltage becomes lower than the Minimum Voltage.
      mask TypeOptions LoadType: Constant Z | constant I | constant P
      mask DialogControl ParameterTabVar0 Prompt: Parameters
      mask DialogControl ParameterTabVar1 Prompt: Type
      mask Display:
      | color('red');
      | A=[-210,-180,-170,-160,-147,-140,-130,-120,-110,-80,-50,-49,-45,-39,-33,-26,-21,-18,-17,-19,-22,-22,-26,-27,-25,-22,-16,-9,-3,2,6,6,4,1,1,-3,-4,-2,2,7,14,20,26,29,30,28,24,24,21,20,21,25,31,37,44,49,50,50,80];
      | B=[-41.5,-41.5,-63,-20,-63,-20,-63,-20,-41.5,-41.5,-41.5,-34,-26,-21,-20,-22,-28,-37,-47,-57,-63,-63,-54,-44,-34,-26,-21,-20,-22,-28,-37,-47,-57,-63,-63,-54,-44,-34,-26,-21,-20,-22,-28,-37,-47,-57,-63,-63,-54,-44,-34,-26,-21,-20,-22,-28,-37,-41.50,-41.5];
      | plot(A,B);
      | color('black');
      | port_label('LConn', 1, '+')
  38-39 10 : powerlib/Elements/Pi Section Line  LConnTagsString=__new0  RConnTagsString=__new0  Frequency=60  Resistance=R1_10  Inductance=L1_10  Capacitance=C1_10  Length=325*ft2km  PiSections=1  Measurements=None
      settings: AttributesFormatString=\n  SourceProductName=Simscape Electrical  SourceProductBaseCode=PS
  39 : Subsystem
  39 Y PQ : Subsystem  mask(Single Phase ZIP Load){Vnom=1.0*2401.78, fnom=60, Pnom=20e3*a, Qnom=10e3*a, LoadType=constant P, Vlim=0.7}
      mask prompts: Vnom "Nominal Voltage Vn (Vrms)"; fnom "Nominal Frequency fn (Hz)"; Pnom "Nominal Active power (W)"; Qnom "Nominal Reactive power (VAR)"; LoadType "Load Type"; Vlim "Minimum voltage (pu)"
      mask help:
      | Notes:
      | Single Phase ZIP load model which gets converted to constant Z type if the voltage becomes lower than the Minimum Voltage.
      mask TypeOptions LoadType: Constant Z | constant I | constant P
      mask DialogControl ParameterTabVar0 Prompt: Parameters
      mask DialogControl ParameterTabVar1 Prompt: Type
      mask Display:
      | color('red');
      | A=[-210,-180,-170,-160,-147,-140,-130,-120,-110,-80,-50,-49,-45,-39,-33,-26,-21,-18,-17,-19,-22,-22,-26,-27,-25,-22,-16,-9,-3,2,6,6,4,1,1,-3,-4,-2,2,7,14,20,26,29,30,28,24,24,21,20,21,25,31,37,44,49,50,50,80];
      | B=[-41.5,-41.5,-63,-20,-63,-20,-63,-20,-41.5,-41.5,-41.5,-34,-26,-21,-20,-22,-28,-37,-47,-57,-63,-63,-54,-44,-34,-26,-21,-20,-22,-28,-37,-47,-57,-63,-63,-54,-44,-34,-26,-21,-20,-22,-28,-37,-47,-57,-63,-63,-54,-44,-34,-26,-21,-20,-22,-28,-37,-41.50,-41.5];
      | plot(A,B);
      | color('black');
      | port_label('LConn', 1, '+')
  4 : Subsystem
  40 : powerlib/Measurements/Three-Phase V-I Measurement  VoltageMeasurement=phase-to-ground  SetLabelV=on  LabelV=V40  Vpu=off  VpuLL=off  CurrentMeasurement=no  SetLabelI=on  LabelI=I800  Ipu=off  Pbase=100e6  Vbase=24900  OutputType=Complex  PhasorSimulation=on  PSBequivalent=0
      settings: SourceProductName=Simscape Electrical
  40-41 11 : powerlib/Elements/Pi Section Line  LConnTagsString=__new0  RConnTagsString=__new0  Frequency=60  Resistance=R1_11  Inductance=L1_11  Capacitance=C1_11  Length=325*ft2km  PiSections=1  Measurements=None
      settings: AttributesFormatString=\n  SourceProductName=Simscape Electrical  SourceProductBaseCode=PS
  40-42 1 : powerlib/Elements/Three-Phase PI Section Line  LConnTagsString=a|b|c  RConnTagsString=A|B|C  Frequency=60  Resistances=[R1_1 R0_1]  Inductances=[L1_1 L0_1]  Capacitances=[C1_1 C0_1]  Length=250*ft2km
      settings: SourceProductName=Simscape Electrical
  41 : Subsystem
  41 Y PQ : Subsystem  mask(Single Phase ZIP Load){Vnom=1.0*2401.78, fnom=60, Pnom=20e3*a, Qnom=10e3*a, LoadType=constant P, Vlim=0.7}
      mask prompts: Vnom "Nominal Voltage Vn (Vrms)"; fnom "Nominal Frequency fn (Hz)"; Pnom "Nominal Active power (W)"; Qnom "Nominal Reactive power (VAR)"; LoadType "Load Type"; Vlim "Minimum voltage (pu)"
      mask help:
      | Notes:
      | Single Phase ZIP load model which gets converted to constant Z type if the voltage becomes lower than the Minimum Voltage.
      mask TypeOptions LoadType: Constant Z | constant I | constant P
      mask DialogControl ParameterTabVar0 Prompt: Parameters
      mask DialogControl ParameterTabVar1 Prompt: Type
      mask Display:
      | color('red');
      | A=[-210,-180,-170,-160,-147,-140,-130,-120,-110,-80,-50,-49,-45,-39,-33,-26,-21,-18,-17,-19,-22,-22,-26,-27,-25,-22,-16,-9,-3,2,6,6,4,1,1,-3,-4,-2,2,7,14,20,26,29,30,28,24,24,21,20,21,25,31,37,44,49,50,50,80];
      | B=[-41.5,-41.5,-63,-20,-63,-20,-63,-20,-41.5,-41.5,-41.5,-34,-26,-21,-20,-22,-28,-37,-47,-57,-63,-63,-54,-44,-34,-26,-21,-20,-22,-28,-37,-47,-57,-63,-63,-54,-44,-34,-26,-21,-20,-22,-28,-37,-47,-57,-63,-63,-54,-44,-34,-26,-21,-20,-22,-28,-37,-41.50,-41.5];
      | plot(A,B);
      | color('black');
      | port_label('LConn', 1, '+')
  4160 V swing : powerlib/Electrical Sources/Three-Phase Source  InternalConnection=Yg  VoltagePhases=on  Voltage=120e3  PhaseAngle=0  Voltage_phases=[1.0 1.0 1.0]*4160/sqrt(3)  PhaseAngles_phases=[0 -120 120 ]  Frequency=60  NonIdealSource=off  SpecifyImpedance=on  Resistance=.0001  Inductance=16.58e-3  ShortCircuitLevel=10e6  BaseVoltage=4160  XRratio=4.67e4  BusType=swing  Pref=0  Qref=0  Prefabc=[4e6/3 4e6/3 4e6/3]  Qrefabc=[0 0 0]  Qmin="[-inf  -inf -inf]"  Qmax="[inf  inf inf]"
      settings: SourceProductName=Simscape Electrical
  42 : powerlib/Measurements/Three-Phase V-I Measurement  VoltageMeasurement=phase-to-ground  SetLabelV=on  LabelV=V42  Vpu=off  VpuLL=off  CurrentMeasurement=no  SetLabelI=on  LabelI=I800  Ipu=off  Pbase=100e6  Vbase=24900  OutputType=Complex  PhasorSimulation=on  PSBequivalent=0
      settings: SourceProductName=Simscape Electrical
  42 Y PQ : Subsystem  mask(Single Phase ZIP Load){Vnom=1.0*2401.78, fnom=60, Pnom=20e3*a, Qnom=10e3*a, LoadType=constant P, Vlim=0.7}
      mask prompts: Vnom "Nominal Voltage Vn (Vrms)"; fnom "Nominal Frequency fn (Hz)"; Pnom "Nominal Active power (W)"; Qnom "Nominal Reactive power (VAR)"; LoadType "Load Type"; Vlim "Minimum voltage (pu)"
      mask help:
      | Notes:
      | Single Phase ZIP load model which gets converted to constant Z type if the voltage becomes lower than the Minimum Voltage.
      mask TypeOptions LoadType: Constant Z | constant I | constant P
      mask DialogControl ParameterTabVar0 Prompt: Parameters
      mask DialogControl ParameterTabVar1 Prompt: Type
      mask Display:
      | color('red');
      | A=[-210,-180,-170,-160,-147,-140,-130,-120,-110,-80,-50,-49,-45,-39,-33,-26,-21,-18,-17,-19,-22,-22,-26,-27,-25,-22,-16,-9,-3,2,6,6,4,1,1,-3,-4,-2,2,7,14,20,26,29,30,28,24,24,21,20,21,25,31,37,44,49,50,50,80];
      | B=[-41.5,-41.5,-63,-20,-63,-20,-63,-20,-41.5,-41.5,-41.5,-34,-26,-21,-20,-22,-28,-37,-47,-57,-63,-63,-54,-44,-34,-26,-21,-20,-22,-28,-37,-47,-57,-63,-63,-54,-44,-34,-26,-21,-20,-22,-28,-37,-47,-57,-63,-63,-54,-44,-34,-26,-21,-20,-22,-28,-37,-41.50,-41.5];
      | plot(A,B);
      | color('black');
      | port_label('LConn', 1, '+')
  42-43 10 : powerlib/Elements/Pi Section Line  LConnTagsString=__new0  RConnTagsString=__new0  Frequency=60  Resistance=R1_10  Inductance=L1_10  Capacitance=C1_10  Length=500*ft2km  PiSections=1  Measurements=None
      settings: AttributesFormatString=\n  SourceProductName=Simscape Electrical  SourceProductBaseCode=PS
  42-44 1 : powerlib/Elements/Three-Phase PI Section Line  LConnTagsString=a|b|c  RConnTagsString=A|B|C  Frequency=60  Resistances=[R1_1 R0_1]  Inductances=[L1_1 L0_1]  Capacitances=[C1_1 C0_1]  Length=200*ft2km
      settings: SourceProductName=Simscape Electrical
  43 : Subsystem
  43 Y Z : Subsystem  mask(Single Phase ZIP Load){Vnom=1.0*2401.78, fnom=60, Pnom=40e3*a, Qnom=20e3*a, LoadType=Constant Z, Vlim=0.7}
      mask prompts: Vnom "Nominal Voltage Vn (Vrms)"; fnom "Nominal Frequency fn (Hz)"; Pnom "Nominal Active power (W)"; Qnom "Nominal Reactive power (VAR)"; LoadType "Load Type"; Vlim "Minimum voltage (pu)"
      mask help:
      | Notes:
      | Single Phase ZIP load model which gets converted to constant Z type if the voltage becomes lower than the Minimum Voltage.
      mask TypeOptions LoadType: Constant Z | constant I | constant P
      mask DialogControl ParameterTabVar0 Prompt: Parameters
      mask DialogControl ParameterTabVar1 Prompt: Type
      mask Display:
      | color('red');
      | A=[-210,-180,-170,-160,-147,-140,-130,-120,-110,-80,-50,-49,-45,-39,-33,-26,-21,-18,-17,-19,-22,-22,-26,-27,-25,-22,-16,-9,-3,2,6,6,4,1,1,-3,-4,-2,2,7,14,20,26,29,30,28,24,24,21,20,21,25,31,37,44,49,50,50,80];
      | B=[-41.5,-41.5,-63,-20,-63,-20,-63,-20,-41.5,-41.5,-41.5,-34,-26,-21,-20,-22,-28,-37,-47,-57,-63,-63,-54,-44,-34,-26,-21,-20,-22,-28,-37,-47,-57,-63,-63,-54,-44,-34,-26,-21,-20,-22,-28,-37,-47,-57,-63,-63,-54,-44,-34,-26,-21,-20,-22,-28,-37,-41.50,-41.5];
      | plot(A,B);
      | color('black');
      | port_label('LConn', 1, '+')
  44 : powerlib/Measurements/Three-Phase V-I Measurement  VoltageMeasurement=phase-to-ground  SetLabelV=on  LabelV=V44  Vpu=off  VpuLL=off  CurrentMeasurement=no  SetLabelI=on  LabelI=I800  Ipu=off  Pbase=100e6  Vbase=24900  OutputType=Complex  PhasorSimulation=on  PSBequivalent=0
      settings: SourceProductName=Simscape Electrical
  44-45 9 : powerlib/Elements/Pi Section Line  LConnTagsString=__new0  RConnTagsString=__new0  Frequency=60  Resistance=R1_9  Inductance=L1_9  Capacitance=C1_9  Length=200*ft2km  PiSections=1  Measurements=None
      settings: AttributesFormatString=\n  SourceProductName=Simscape Electrical  SourceProductBaseCode=PS
  44-47 1 : powerlib/Elements/Three-Phase PI Section Line  LConnTagsString=a|b|c  RConnTagsString=A|B|C  Frequency=60  Resistances=[R1_1 R0_1]  Inductances=[L1_1 L0_1]  Capacitances=[C1_1 C0_1]  Length=250*ft2km
      settings: SourceProductName=Simscape Electrical
  45 : Subsystem
  45 Y I : Subsystem  mask(Single Phase ZIP Load){Vnom=1.0*2401.78, fnom=60, Pnom=20e3*a, Qnom=10e3*a, LoadType=constant I, Vlim=0.7}
      mask prompts: Vnom "Nominal Voltage Vn (Vrms)"; fnom "Nominal Frequency fn (Hz)"; Pnom "Nominal Active power (W)"; Qnom "Nominal Reactive power (VAR)"; LoadType "Load Type"; Vlim "Minimum voltage (pu)"
      mask help:
      | Notes:
      | Single Phase ZIP load model which gets converted to constant Z type if the voltage becomes lower than the Minimum Voltage.
      mask TypeOptions LoadType: Constant Z | constant I | constant P
      mask DialogControl ParameterTabVar0 Prompt: Parameters
      mask DialogControl ParameterTabVar1 Prompt: Type
      mask Display:
      | color('red');
      | A=[-210,-180,-170,-160,-147,-140,-130,-120,-110,-80,-50,-49,-45,-39,-33,-26,-21,-18,-17,-19,-22,-22,-26,-27,-25,-22,-16,-9,-3,2,6,6,4,1,1,-3,-4,-2,2,7,14,20,26,29,30,28,24,24,21,20,21,25,31,37,44,49,50,50,80];
      | B=[-41.5,-41.5,-63,-20,-63,-20,-63,-20,-41.5,-41.5,-41.5,-34,-26,-21,-20,-22,-28,-37,-47,-57,-63,-63,-54,-44,-34,-26,-21,-20,-22,-28,-37,-47,-57,-63,-63,-54,-44,-34,-26,-21,-20,-22,-28,-37,-47,-57,-63,-63,-54,-44,-34,-26,-21,-20,-22,-28,-37,-41.50,-41.5];
      | plot(A,B);
      | color('black');
      | port_label('LConn', 1, '+')
  45-46 9 : powerlib/Elements/Pi Section Line  LConnTagsString=__new0  RConnTagsString=__new0  Frequency=60  Resistance=R1_9  Inductance=L1_9  Capacitance=C1_9  Length=300*ft2km  PiSections=1  Measurements=None
      settings: AttributesFormatString=\n  SourceProductName=Simscape Electrical  SourceProductBaseCode=PS
  450 : powerlib/Measurements/Three-Phase V-I Measurement  VoltageMeasurement=phase-to-ground  SetLabelV=on  LabelV=V450  Vpu=off  VpuLL=off  CurrentMeasurement=no  SetLabelI=on  LabelI=I65  Ipu=off  Pbase=100e6  Vbase=24900  OutputType=Complex  PhasorSimulation=on  PSBequivalent=0
      settings: SourceProductName=Simscape Electrical
  450-451 : powerlib/Elements/Three-Phase Breaker  InitialState=open  SwitchA=off  SwitchB=off  SwitchC=off  SwitchTimes="[1/60  5/60]"  External=off  BreakerResistance=1e-6  SnubberResistance=1e6  SnubberCapacitance=inf  Measurements=None
      settings: SourceProductName=Simscape Electrical
  46 : Subsystem
  46 Y PQ : Subsystem  mask(Single Phase ZIP Load){Vnom=1.0*2401.78, fnom=60, Pnom=20e3*a, Qnom=10e3*a, LoadType=constant P, Vlim=0.7}
      mask prompts: Vnom "Nominal Voltage Vn (Vrms)"; fnom "Nominal Frequency fn (Hz)"; Pnom "Nominal Active power (W)"; Qnom "Nominal Reactive power (VAR)"; LoadType "Load Type"; Vlim "Minimum voltage (pu)"
      mask help:
      | Notes:
      | Single Phase ZIP load model which gets converted to constant Z type if the voltage becomes lower than the Minimum Voltage.
      mask TypeOptions LoadType: Constant Z | constant I | constant P
      mask DialogControl ParameterTabVar0 Prompt: Parameters
      mask DialogControl ParameterTabVar1 Prompt: Type
      mask Display:
      | color('red');
      | A=[-210,-180,-170,-160,-147,-140,-130,-120,-110,-80,-50,-49,-45,-39,-33,-26,-21,-18,-17,-19,-22,-22,-26,-27,-25,-22,-16,-9,-3,2,6,6,4,1,1,-3,-4,-2,2,7,14,20,26,29,30,28,24,24,21,20,21,25,31,37,44,49,50,50,80];
      | B=[-41.5,-41.5,-63,-20,-63,-20,-63,-20,-41.5,-41.5,-41.5,-34,-26,-21,-20,-22,-28,-37,-47,-57,-63,-63,-54,-44,-34,-26,-21,-20,-22,-28,-37,-47,-57,-63,-63,-54,-44,-34,-26,-21,-20,-22,-28,-37,-47,-57,-63,-63,-54,-44,-34,-26,-21,-20,-22,-28,-37,-41.50,-41.5];
      | plot(A,B);
      | color('black');
      | port_label('LConn', 1, '+')
  47 : powerlib/Measurements/Three-Phase V-I Measurement  VoltageMeasurement=phase-to-ground  SetLabelV=on  LabelV=V47  Vpu=off  VpuLL=off  CurrentMeasurement=no  SetLabelI=on  LabelI=I800  Ipu=off  Pbase=100e6  Vbase=24900  OutputType=Complex  PhasorSimulation=on  PSBequivalent=0
      settings: SourceProductName=Simscape Electrical
  47 Y I : Subsystem  mask(Three Phase Star ZIP Load (Phasor)){Vnom=4160, fnom=60, Pnom=[35 35 35 ]*1e3*a, Qnom=[25 25 25 ]*1e3*a, LoadType=Constant I, Vlim=0.7}
      mask prompts: Vnom "Nominal Ph-Ph voltage (Vrms)"; fnom "Nominal Frequency fn (Hz)"; Pnom "Nominal Per Phase Active Power [Pa Pb Pc] (W)"; Qnom "Nominal Per Phase Reactive Power [Qa Qb Qc] (VAR)"; LoadType "Load Type"; Vlim "Minimum voltage (pu)"
      mask help:
      | Notes:
      | Three Phase Star Connected ZIP load model which gets converted to constant Z type if the voltage becomes lower than the Minimum Voltage.
      mask TypeOptions LoadType: Constant Z | Constant I | Constant P
      mask DialogControl ParameterTabVar0 Prompt: Parameters
      mask DialogControl ParameterTabVar01 Prompt: Type
      mask Display:
      | color('red');
      | %load figure 0deg
      | A=[-210,-180,-170,-160,-147,-140,-130,-120,-110,-80,-50,-49,-45,-39,-33,-26,-21,-18,-17,-19,-22,-22,-26,-27,-25,-22,-16,-9,-3,2,6,6,4,1,1,-3,-4,-2,2,7,14,20,26,29,30,28,24,24,21,20,21,25,31,37,44,49,50,50,80];
      | B=[-41.5,-41.5,-63,-20,-63,-20,-63,-20,-41.5,-41.5,-41.5,-34,-26,-21,-20,-22,-28,-37,-47,-57,-63,-63,-54,-44,-34,-26,-21,-20,-22,-28,-37,-47,-57,-63,-63,-54,-44,-34,-26,-21,-20,-22,-28,-37,-47,-57,-63,-63,-54,-44,-34,-26,-21,-20,-22,-28,-37,-41.50,-41.5];
      | % plot(A,B);
      | 
      | %load figure 0deg inverted
      | A1=[-80,-50,-49,-45,-39,-33,-26,-21,-18,-17,-19,-22,-22,-26,-27,-25,-22,-16,-9,-3,2,6,6,4,1,1,-3,-4,-2,2,7,14,20,26,29,30,28,24,24,21,20,21,25,31,37,44,49,50,50,80,110,120,130,143,150,160,170,180,210];
      | B1=[-41.5,-41.5,-34,-26,-21,-20,-22,-28,-37,-47,-57,-63,-63,-54,-44,-34,-26,-21,-20,-22,-28,-37,-47,-57,-63,-63,-54,-44,-34,-26,-21,-20,-22,-28,-37,-47,-57,-63,-63,-54,-44,-34,-26,-21,-20,-22,-28,-37,-41.5,-41.5,-41.5,-63,-20,-63,-20,-63,-20,-41.5,-41.5];
      | 
      | 
      | %load figure 90deg
      | C=[-41.5,-41.5,-20,-63,-20,-63,-20,-63,-41.5,-41.5,-41.5,-37,-28,-22,-20,-21,-26,-34,-44,-54,-63,-63,-57,-47,-37,-28,-22,-20,-21,-26,-34,-44,-54,-63,-63,-57,-47,-37,-28,-22,-20,-21,-26,-34,-44,-54,-63,-63,-57,-47,-37,-28,-22,-20,-21,-26,-34,-41.5,-41.5];
      | D=[190,160,150,140,130,123,110,100,90,80,50,50,49,44,37,31,25,21,20,21,24,24,28,30,29,26,20,14,7,2,-2,-4,-3,1,1,4,6,6,2,-3,-9,-16,-22,-25,-27,-26,-22,-22,-19,-17,-18,-21,-26,-33,-39,-45,-49,-50,-70];
      | plot(C,D);
      | 
      | 
      | %load figure -120deg
      | c=1*exp(sqrt(-1)*(-60*pi/180));
      | l=A1+j*B1;
      | m=l*c;
      | E=real(m);F=imag(m);
      | E=E+34.4400;F=F-118.53;
      | plot(E,F);
      | 
      | %load figure +120deg
      | c=1*exp(sqrt(-1)*(60*pi/180));
      | l=A+j*B;
      | m=l*c;
      | G=real(m);
      | H=imag(m);
      | G=G-117.44;H=H-118.5300;
      | plot(G,H);
      | 
      | color('black');
      | port_label('LConn', 1, 'A')
      | port_label('LConn', 2, 'B')
      | port_label('LConn', 3, 'C')
  47-48 4 : powerlib/Elements/Three-Phase PI Section Line  LConnTagsString=a|b|c  RConnTagsString=A|B|C  Frequency=60  Resistances=[R1_4 R0_4]  Inductances=[L1_4 L0_4]  Capacitances=[C1_4 C0_4]  Length=150*ft2km
      settings: SourceProductName=Simscape Electrical
  47-49 4 : powerlib/Elements/Three-Phase PI Section Line  LConnTagsString=a|b|c  RConnTagsString=A|B|C  Frequency=60  Resistances=[R1_4 R0_4]  Inductances=[L1_4 L0_4]  Capacitances=[C1_4 C0_4]  Length=250*ft2km
      settings: SourceProductName=Simscape Electrical
  48 : powerlib/Measurements/Three-Phase V-I Measurement  VoltageMeasurement=phase-to-ground  SetLabelV=on  LabelV=V48  Vpu=off  VpuLL=off  CurrentMeasurement=no  SetLabelI=on  LabelI=I800  Ipu=off  Pbase=100e6  Vbase=24900  OutputType=Complex  PhasorSimulation=on  PSBequivalent=0
      settings: SourceProductName=Simscape Electrical
  48 Y Z : Subsystem  mask(Three Phase Star ZIP Load (Phasor)){Vnom=4160, fnom=60, Pnom=[70 70 70]*1e3*a, Qnom=[50 50 50]*1e3*a, LoadType=Constant Z, Vlim=0.7}
      mask prompts: Vnom "Nominal Ph-Ph voltage (Vrms)"; fnom "Nominal Frequency fn (Hz)"; Pnom "Nominal Per Phase Active Power [Pa Pb Pc] (W)"; Qnom "Nominal Per Phase Reactive Power [Qa Qb Qc] (VAR)"; LoadType "Load Type"; Vlim "Minimum voltage (pu)"
      mask help:
      | Notes:
      | Three Phase Star Connected ZIP load model which gets converted to constant Z type if the voltage becomes lower than the Minimum Voltage.
      mask TypeOptions LoadType: Constant Z | Constant I | Constant P
      mask DialogControl ParameterTabVar0 Prompt: Parameters
      mask DialogControl ParameterTabVar01 Prompt: Type
      mask Display:
      | color('red');
      | %load figure 0deg
      | A=[-210,-180,-170,-160,-147,-140,-130,-120,-110,-80,-50,-49,-45,-39,-33,-26,-21,-18,-17,-19,-22,-22,-26,-27,-25,-22,-16,-9,-3,2,6,6,4,1,1,-3,-4,-2,2,7,14,20,26,29,30,28,24,24,21,20,21,25,31,37,44,49,50,50,80];
      | B=[-41.5,-41.5,-63,-20,-63,-20,-63,-20,-41.5,-41.5,-41.5,-34,-26,-21,-20,-22,-28,-37,-47,-57,-63,-63,-54,-44,-34,-26,-21,-20,-22,-28,-37,-47,-57,-63,-63,-54,-44,-34,-26,-21,-20,-22,-28,-37,-47,-57,-63,-63,-54,-44,-34,-26,-21,-20,-22,-28,-37,-41.50,-41.5];
      | % plot(A,B);
      | 
      | %load figure 0deg inverted
      | A1=[-80,-50,-49,-45,-39,-33,-26,-21,-18,-17,-19,-22,-22,-26,-27,-25,-22,-16,-9,-3,2,6,6,4,1,1,-3,-4,-2,2,7,14,20,26,29,30,28,24,24,21,20,21,25,31,37,44,49,50,50,80,110,120,130,143,150,160,170,180,210];
      | B1=[-41.5,-41.5,-34,-26,-21,-20,-22,-28,-37,-47,-57,-63,-63,-54,-44,-34,-26,-21,-20,-22,-28,-37,-47,-57,-63,-63,-54,-44,-34,-26,-21,-20,-22,-28,-37,-47,-57,-63,-63,-54,-44,-34,-26,-21,-20,-22,-28,-37,-41.5,-41.5,-41.5,-63,-20,-63,-20,-63,-20,-41.5,-41.5];
      | 
      | 
      | %load figure 90deg
      | C=[-41.5,-41.5,-20,-63,-20,-63,-20,-63,-41.5,-41.5,-41.5,-37,-28,-22,-20,-21,-26,-34,-44,-54,-63,-63,-57,-47,-37,-28,-22,-20,-21,-26,-34,-44,-54,-63,-63,-57,-47,-37,-28,-22,-20,-21,-26,-34,-44,-54,-63,-63,-57,-47,-37,-28,-22,-20,-21,-26,-34,-41.5,-41.5];
      | D=[190,160,150,140,130,123,110,100,90,80,50,50,49,44,37,31,25,21,20,21,24,24,28,30,29,26,20,14,7,2,-2,-4,-3,1,1,4,6,6,2,-3,-9,-16,-22,-25,-27,-26,-22,-22,-19,-17,-18,-21,-26,-33,-39,-45,-49,-50,-70];
      | plot(C,D);
      | 
      | 
      | %load figure -120deg
      | c=1*exp(sqrt(-1)*(-60*pi/180));
      | l=A1+j*B1;
      | m=l*c;
      | E=real(m);F=imag(m);
      | E=E+34.4400;F=F-118.53;
      | plot(E,F);
      | 
      | %load figure +120deg
      | c=1*exp(sqrt(-1)*(60*pi/180));
      | l=A+j*B;
      | m=l*c;
      | G=real(m);
      | H=imag(m);
      | G=G-117.44;H=H-118.5300;
      | plot(G,H);
      | 
      | color('black');
      | port_label('LConn', 1, 'A')
      | port_label('LConn', 2, 'B')
      | port_label('LConn', 3, 'C')
  49 : powerlib/Measurements/Three-Phase V-I Measurement  VoltageMeasurement=phase-to-ground  SetLabelV=on  LabelV=V49  Vpu=off  VpuLL=off  CurrentMeasurement=no  SetLabelI=on  LabelI=I800  Ipu=off  Pbase=100e6  Vbase=24900  OutputType=Complex  PhasorSimulation=on  PSBequivalent=0
      settings: SourceProductName=Simscape Electrical
  49 Y PQ : Subsystem  mask(Three Phase Star ZIP Load (Phasor)){Vnom=4160, fnom=60, Pnom=[35 70 35]*1e3*a, Qnom=[25 50 20]*1e3*a, LoadType=Constant P, Vlim=0.7}
      mask prompts: Vnom "Nominal Ph-Ph voltage (Vrms)"; fnom "Nominal Frequency fn (Hz)"; Pnom "Nominal Per Phase Active Power [Pa Pb Pc] (W)"; Qnom "Nominal Per Phase Reactive Power [Qa Qb Qc] (VAR)"; LoadType "Load Type"; Vlim "Minimum voltage (pu)"
      mask help:
      | Notes:
      | Three Phase Star Connected ZIP load model which gets converted to constant Z type if the voltage becomes lower than the Minimum Voltage.
      mask TypeOptions LoadType: Constant Z | Constant I | Constant P
      mask DialogControl ParameterTabVar0 Prompt: Parameters
      mask DialogControl ParameterTabVar01 Prompt: Type
      mask Display:
      | color('red');
      | %load figure 0deg
      | A=[-210,-180,-170,-160,-147,-140,-130,-120,-110,-80,-50,-49,-45,-39,-33,-26,-21,-18,-17,-19,-22,-22,-26,-27,-25,-22,-16,-9,-3,2,6,6,4,1,1,-3,-4,-2,2,7,14,20,26,29,30,28,24,24,21,20,21,25,31,37,44,49,50,50,80];
      | B=[-41.5,-41.5,-63,-20,-63,-20,-63,-20,-41.5,-41.5,-41.5,-34,-26,-21,-20,-22,-28,-37,-47,-57,-63,-63,-54,-44,-34,-26,-21,-20,-22,-28,-37,-47,-57,-63,-63,-54,-44,-34,-26,-21,-20,-22,-28,-37,-47,-57,-63,-63,-54,-44,-34,-26,-21,-20,-22,-28,-37,-41.50,-41.5];
      | % plot(A,B);
      | 
      | %load figure 0deg inverted
      | A1=[-80,-50,-49,-45,-39,-33,-26,-21,-18,-17,-19,-22,-22,-26,-27,-25,-22,-16,-9,-3,2,6,6,4,1,1,-3,-4,-2,2,7,14,20,26,29,30,28,24,24,21,20,21,25,31,37,44,49,50,50,80,110,120,130,143,150,160,170,180,210];
      | B1=[-41.5,-41.5,-34,-26,-21,-20,-22,-28,-37,-47,-57,-63,-63,-54,-44,-34,-26,-21,-20,-22,-28,-37,-47,-57,-63,-63,-54,-44,-34,-26,-21,-20,-22,-28,-37,-47,-57,-63,-63,-54,-44,-34,-26,-21,-20,-22,-28,-37,-41.5,-41.5,-41.5,-63,-20,-63,-20,-63,-20,-41.5,-41.5];
      | 
      | 
      | %load figure 90deg
      | C=[-41.5,-41.5,-20,-63,-20,-63,-20,-63,-41.5,-41.5,-41.5,-37,-28,-22,-20,-21,-26,-34,-44,-54,-63,-63,-57,-47,-37,-28,-22,-20,-21,-26,-34,-44,-54,-63,-63,-57,-47,-37,-28,-22,-20,-21,-26,-34,-44,-54,-63,-63,-57,-47,-37,-28,-22,-20,-21,-26,-34,-41.5,-41.5];
      | D=[190,160,150,140,130,123,110,100,90,80,50,50,49,44,37,31,25,21,20,21,24,24,28,30,29,26,20,14,7,2,-2,-4,-3,1,1,4,6,6,2,-3,-9,-16,-22,-25,-27,-26,-22,-22,-19,-17,-18,-21,-26,-33,-39,-45,-49,-50,-70];
      | plot(C,D);
      | 
      | 
      | %load figure -120deg
      | c=1*exp(sqrt(-1)*(-60*pi/180));
      | l=A1+j*B1;
      | m=l*c;
      | E=real(m);F=imag(m);
      | E=E+34.4400;F=F-118.53;
      | plot(E,F);
      | 
      | %load figure +120deg
      | c=1*exp(sqrt(-1)*(60*pi/180));
      | l=A+j*B;
      | m=l*c;
      | G=real(m);
      | H=imag(m);
      | G=G-117.44;H=H-118.5300;
      | plot(G,H);
      | 
      | color('black');
      | port_label('LConn', 1, 'A')
      | port_label('LConn', 2, 'B')
      | port_label('LConn', 3, 'C')
  49-50 4 : powerlib/Elements/Three-Phase PI Section Line  LConnTagsString=a|b|c  RConnTagsString=A|B|C  Frequency=60  Resistances=[R1_4 R0_4]  Inductances=[L1_4 L0_4]  Capacitances=[C1_4 C0_4]  Length=250*ft2km
      settings: SourceProductName=Simscape Electrical
  4Y PQ : Subsystem  mask(Single Phase ZIP Load){Vnom=1.0*2401.78, fnom=60, Pnom=40e3*a, Qnom=20e3*a, LoadType=constant P, Vlim=0.7}
      mask prompts: Vnom "Nominal Voltage Vn (Vrms)"; fnom "Nominal Frequency fn (Hz)"; Pnom "Nominal Active power (W)"; Qnom "Nominal Reactive power (VAR)"; LoadType "Load Type"; Vlim "Minimum voltage (pu)"
      mask help:
      | Notes:
      | Single Phase ZIP load model which gets converted to constant Z type if the voltage becomes lower than the Minimum Voltage.
      mask TypeOptions LoadType: Constant Z | constant I | constant P
      mask DialogControl ParameterTabVar0 Prompt: Parameters
      mask DialogControl ParameterTabVar1 Prompt: Type
      mask Display:
      | color('red');
      | A=[-210,-180,-170,-160,-147,-140,-130,-120,-110,-80,-50,-49,-45,-39,-33,-26,-21,-18,-17,-19,-22,-22,-26,-27,-25,-22,-16,-9,-3,2,6,6,4,1,1,-3,-4,-2,2,7,14,20,26,29,30,28,24,24,21,20,21,25,31,37,44,49,50,50,80];
      | B=[-41.5,-41.5,-63,-20,-63,-20,-63,-20,-41.5,-41.5,-41.5,-34,-26,-21,-20,-22,-28,-37,-47,-57,-63,-63,-54,-44,-34,-26,-21,-20,-22,-28,-37,-47,-57,-63,-63,-54,-44,-34,-26,-21,-20,-22,-28,-37,-47,-57,-63,-63,-54,-44,-34,-26,-21,-20,-22,-28,-37,-41.50,-41.5];
      | plot(A,B);
      | color('black');
      | port_label('LConn', 1, '+')
  5 : Subsystem
  5 Y I : Subsystem  mask(Single Phase ZIP Load){Vnom=1.0*2401.78, fnom=60, Pnom=20e3*a, Qnom=10e3*a, LoadType=constant I, Vlim=0.7}
      mask prompts: Vnom "Nominal Voltage Vn (Vrms)"; fnom "Nominal Frequency fn (Hz)"; Pnom "Nominal Active power (W)"; Qnom "Nominal Reactive power (VAR)"; LoadType "Load Type"; Vlim "Minimum voltage (pu)"
      mask help:
      | Notes:
      | Single Phase ZIP load model which gets converted to constant Z type if the voltage becomes lower than the Minimum Voltage.
      mask TypeOptions LoadType: Constant Z | constant I | constant P
      mask DialogControl ParameterTabVar0 Prompt: Parameters
      mask DialogControl ParameterTabVar1 Prompt: Type
      mask Display:
      | color('red');
      | A=[-210,-180,-170,-160,-147,-140,-130,-120,-110,-80,-50,-49,-45,-39,-33,-26,-21,-18,-17,-19,-22,-22,-26,-27,-25,-22,-16,-9,-3,2,6,6,4,1,1,-3,-4,-2,2,7,14,20,26,29,30,28,24,24,21,20,21,25,31,37,44,49,50,50,80];
      | B=[-41.5,-41.5,-63,-20,-63,-20,-63,-20,-41.5,-41.5,-41.5,-34,-26,-21,-20,-22,-28,-37,-47,-57,-63,-63,-54,-44,-34,-26,-21,-20,-22,-28,-37,-47,-57,-63,-63,-54,-44,-34,-26,-21,-20,-22,-28,-37,-47,-57,-63,-63,-54,-44,-34,-26,-21,-20,-22,-28,-37,-41.50,-41.5];
      | plot(A,B);
      | color('black');
      | port_label('LConn', 1, '+')
  5-6 11 : powerlib/Elements/Pi Section Line  LConnTagsString=__new0  RConnTagsString=__new0  Frequency=60  Resistance=R1_11  Inductance=L1_11  Capacitance=C1_11  Length=250*ft2km  PiSections=1  Measurements=None
      settings: AttributesFormatString=\n  SourceProductName=Simscape Electrical  SourceProductBaseCode=PS
  50 : powerlib/Measurements/Three-Phase V-I Measurement  VoltageMeasurement=phase-to-ground  SetLabelV=on  LabelV=V50  Vpu=off  VpuLL=off  CurrentMeasurement=no  SetLabelI=on  LabelI=I800  Ipu=off  Pbase=100e6  Vbase=24900  OutputType=Complex  PhasorSimulation=on  PSBequivalent=0
      settings: SourceProductName=Simscape Electrical
  50 Y PQ : Subsystem  mask(Single Phase ZIP Load){Vnom=1.0*2401.78, fnom=60, Pnom=40e3*a, Qnom=20e3*a, LoadType=constant P, Vlim=0.7}
      mask prompts: Vnom "Nominal Voltage Vn (Vrms)"; fnom "Nominal Frequency fn (Hz)"; Pnom "Nominal Active power (W)"; Qnom "Nominal Reactive power (VAR)"; LoadType "Load Type"; Vlim "Minimum voltage (pu)"
      mask help:
      | Notes:
      | Single Phase ZIP load model which gets converted to constant Z type if the voltage becomes lower than the Minimum Voltage.
      mask TypeOptions LoadType: Constant Z | constant I | constant P
      mask DialogControl ParameterTabVar0 Prompt: Parameters
      mask DialogControl ParameterTabVar1 Prompt: Type
      mask Display:
      | color('red');
      | A=[-210,-180,-170,-160,-147,-140,-130,-120,-110,-80,-50,-49,-45,-39,-33,-26,-21,-18,-17,-19,-22,-22,-26,-27,-25,-22,-16,-9,-3,2,6,6,4,1,1,-3,-4,-2,2,7,14,20,26,29,30,28,24,24,21,20,21,25,31,37,44,49,50,50,80];
      | B=[-41.5,-41.5,-63,-20,-63,-20,-63,-20,-41.5,-41.5,-41.5,-34,-26,-21,-20,-22,-28,-37,-47,-57,-63,-63,-54,-44,-34,-26,-21,-20,-22,-28,-37,-47,-57,-63,-63,-54,-44,-34,-26,-21,-20,-22,-28,-37,-47,-57,-63,-63,-54,-44,-34,-26,-21,-20,-22,-28,-37,-41.50,-41.5];
      | plot(A,B);
      | color('black');
      | port_label('LConn', 1, '+')
  50-51 4 : powerlib/Elements/Three-Phase PI Section Line  LConnTagsString=a|b|c  RConnTagsString=A|B|C  Frequency=60  Resistances=[R1_4 R0_4]  Inductances=[L1_4 L0_4]  Capacitances=[C1_4 C0_4]  Length=250*ft2km
      settings: SourceProductName=Simscape Electrical
  51 : powerlib/Measurements/Three-Phase V-I Measurement  VoltageMeasurement=phase-to-ground  SetLabelV=on  LabelV=V51  Vpu=off  VpuLL=off  CurrentMeasurement=no  SetLabelI=on  LabelI=I800  Ipu=off  Pbase=100e6  Vbase=24900  OutputType=Complex  PhasorSimulation=on  PSBequivalent=0
      settings: SourceProductName=Simscape Electrical
  51 Y PQ : Subsystem  mask(Single Phase ZIP Load){Vnom=1.0*2401.78, fnom=60, Pnom=20e3*a, Qnom=10e3*a, LoadType=constant P, Vlim=0.7}
      mask prompts: Vnom "Nominal Voltage Vn (Vrms)"; fnom "Nominal Frequency fn (Hz)"; Pnom "Nominal Active power (W)"; Qnom "Nominal Reactive power (VAR)"; LoadType "Load Type"; Vlim "Minimum voltage (pu)"
      mask help:
      | Notes:
      | Single Phase ZIP load model which gets converted to constant Z type if the voltage becomes lower than the Minimum Voltage.
      mask TypeOptions LoadType: Constant Z | constant I | constant P
      mask DialogControl ParameterTabVar0 Prompt: Parameters
      mask DialogControl ParameterTabVar1 Prompt: Type
      mask Display:
      | color('red');
      | A=[-210,-180,-170,-160,-147,-140,-130,-120,-110,-80,-50,-49,-45,-39,-33,-26,-21,-18,-17,-19,-22,-22,-26,-27,-25,-22,-16,-9,-3,2,6,6,4,1,1,-3,-4,-2,2,7,14,20,26,29,30,28,24,24,21,20,21,25,31,37,44,49,50,50,80];
      | B=[-41.5,-41.5,-63,-20,-63,-20,-63,-20,-41.5,-41.5,-41.5,-34,-26,-21,-20,-22,-28,-37,-47,-57,-63,-63,-54,-44,-34,-26,-21,-20,-22,-28,-37,-47,-57,-63,-63,-54,-44,-34,-26,-21,-20,-22,-28,-37,-47,-57,-63,-63,-54,-44,-34,-26,-21,-20,-22,-28,-37,-41.50,-41.5];
      | plot(A,B);
      | color('black');
      | port_label('LConn', 1, '+')
  51-151 4 : powerlib/Elements/Three-Phase PI Section Line  LConnTagsString=a|b|c  RConnTagsString=A|B|C  Frequency=60  Resistances=[R1_4 R0_4]  Inductances=[L1_4 L0_4]  Capacitances=[C1_4 C0_4]  Length=500*ft2km
      settings: SourceProductName=Simscape Electrical
  52 : powerlib/Measurements/Three-Phase V-I Measurement  VoltageMeasurement=phase-to-ground  SetLabelV=on  LabelV=V52  Vpu=off  VpuLL=off  CurrentMeasurement=no  SetLabelI=on  LabelI=I65  Ipu=off  Pbase=100e6  Vbase=24900  OutputType=Complex  PhasorSimulation=on  PSBequivalent=0
      settings: SourceProductName=Simscape Electrical
  52 Y PQ : Subsystem  mask(Single Phase ZIP Load){Vnom=1.0*2401.78, fnom=60, Pnom=40e3*a, Qnom=20e3*a, LoadType=constant P, Vlim=0.7}
      mask prompts: Vnom "Nominal Voltage Vn (Vrms)"; fnom "Nominal Frequency fn (Hz)"; Pnom "Nominal Active power (W)"; Qnom "Nominal Reactive power (VAR)"; LoadType "Load Type"; Vlim "Minimum voltage (pu)"
      mask help:
      | Notes:
      | Single Phase ZIP load model which gets converted to constant Z type if the voltage becomes lower than the Minimum Voltage.
      mask TypeOptions LoadType: Constant Z | constant I | constant P
      mask DialogControl ParameterTabVar0 Prompt: Parameters
      mask DialogControl ParameterTabVar1 Prompt: Type
      mask Display:
      | color('red');
      | A=[-210,-180,-170,-160,-147,-140,-130,-120,-110,-80,-50,-49,-45,-39,-33,-26,-21,-18,-17,-19,-22,-22,-26,-27,-25,-22,-16,-9,-3,2,6,6,4,1,1,-3,-4,-2,2,7,14,20,26,29,30,28,24,24,21,20,21,25,31,37,44,49,50,50,80];
      | B=[-41.5,-41.5,-63,-20,-63,-20,-63,-20,-41.5,-41.5,-41.5,-34,-26,-21,-20,-22,-28,-37,-47,-57,-63,-63,-54,-44,-34,-26,-21,-20,-22,-28,-37,-47,-57,-63,-63,-54,-44,-34,-26,-21,-20,-22,-28,-37,-47,-57,-63,-63,-54,-44,-34,-26,-21,-20,-22,-28,-37,-41.50,-41.5];
      | plot(A,B);
      | color('black');
      | port_label('LConn', 1, '+')
  52-53 1 : powerlib/Elements/Three-Phase PI Section Line  LConnTagsString=a|b|c  RConnTagsString=A|B|C  Frequency=60  Resistances=[R1_1 R0_1]  Inductances=[L1_1 L0_1]  Capacitances=[C1_1 C0_1]  Length=200*ft2km
      settings: SourceProductName=Simscape Electrical
  53 : powerlib/Measurements/Three-Phase V-I Measurement  VoltageMeasurement=phase-to-ground  SetLabelV=on  LabelV=V53  Vpu=off  VpuLL=off  CurrentMeasurement=no  SetLabelI=on  LabelI=I65  Ipu=off  Pbase=100e6  Vbase=24900  OutputType=Complex  PhasorSimulation=on  PSBequivalent=0
      settings: SourceProductName=Simscape Electrical
  53 Y PQ : Subsystem  mask(Single Phase ZIP Load){Vnom=1.0*2401.78, fnom=60, Pnom=40e3*a, Qnom=20e3*a, LoadType=constant P, Vlim=0.7}
      mask prompts: Vnom "Nominal Voltage Vn (Vrms)"; fnom "Nominal Frequency fn (Hz)"; Pnom "Nominal Active power (W)"; Qnom "Nominal Reactive power (VAR)"; LoadType "Load Type"; Vlim "Minimum voltage (pu)"
      mask help:
      | Notes:
      | Single Phase ZIP load model which gets converted to constant Z type if the voltage becomes lower than the Minimum Voltage.
      mask TypeOptions LoadType: Constant Z | constant I | constant P
      mask DialogControl ParameterTabVar0 Prompt: Parameters
      mask DialogControl ParameterTabVar1 Prompt: Type
      mask Display:
      | color('red');
      | A=[-210,-180,-170,-160,-147,-140,-130,-120,-110,-80,-50,-49,-45,-39,-33,-26,-21,-18,-17,-19,-22,-22,-26,-27,-25,-22,-16,-9,-3,2,6,6,4,1,1,-3,-4,-2,2,7,14,20,26,29,30,28,24,24,21,20,21,25,31,37,44,49,50,50,80];
      | B=[-41.5,-41.5,-63,-20,-63,-20,-63,-20,-41.5,-41.5,-41.5,-34,-26,-21,-20,-22,-28,-37,-47,-57,-63,-63,-54,-44,-34,-26,-21,-20,-22,-28,-37,-47,-57,-63,-63,-54,-44,-34,-26,-21,-20,-22,-28,-37,-47,-57,-63,-63,-54,-44,-34,-26,-21,-20,-22,-28,-37,-41.50,-41.5];
      | plot(A,B);
      | color('black');
      | port_label('LConn', 1, '+')
  53-54 1 : powerlib/Elements/Three-Phase PI Section Line  LConnTagsString=a|b|c  RConnTagsString=A|B|C  Frequency=60  Resistances=[R1_1 R0_1]  Inductances=[L1_1 L0_1]  Capacitances=[C1_1 C0_1]  Length=125*ft2km
      settings: SourceProductName=Simscape Electrical
  54 : powerlib/Measurements/Three-Phase V-I Measurement  VoltageMeasurement=phase-to-ground  SetLabelV=on  LabelV=V54  Vpu=off  VpuLL=off  CurrentMeasurement=no  SetLabelI=on  LabelI=I65  Ipu=off  Pbase=100e6  Vbase=24900  OutputType=Complex  PhasorSimulation=on  PSBequivalent=0
      settings: SourceProductName=Simscape Electrical
  54-55 1 : powerlib/Elements/Three-Phase PI Section Line  LConnTagsString=a|b|c  RConnTagsString=A|B|C  Frequency=60  Resistances=[R1_1 R0_1]  Inductances=[L1_1 L0_1]  Capacitances=[C1_1 C0_1]  Length=275*ft2km
      settings: SourceProductName=Simscape Electrical
  54-57 3 : powerlib/Elements/Three-Phase PI Section Line  LConnTagsString=a|b|c  RConnTagsString=A|B|C  Frequency=60  Resistances=[R1_3 R0_3]  Inductances=[L1_3 L0_3]  Capacitances=[C1_3 C0_3]  Length=350*ft2km
      settings: SourceProductName=Simscape Electrical
  55 : powerlib/Measurements/Three-Phase V-I Measurement  VoltageMeasurement=phase-to-ground  SetLabelV=on  LabelV=V55  Vpu=off  VpuLL=off  CurrentMeasurement=no  SetLabelI=on  LabelI=I65  Ipu=off  Pbase=100e6  Vbase=24900  OutputType=Complex  PhasorSimulation=on  PSBequivalent=0
      settings: SourceProductName=Simscape Electrical
  55 Y Z : Subsystem  mask(Single Phase ZIP Load){Vnom=1.0*2401.78, fnom=60, Pnom=20e3*a, Qnom=10e3*a, LoadType=Constant Z, Vlim=0.7}
      mask prompts: Vnom "Nominal Voltage Vn (Vrms)"; fnom "Nominal Frequency fn (Hz)"; Pnom "Nominal Active power (W)"; Qnom "Nominal Reactive power (VAR)"; LoadType "Load Type"; Vlim "Minimum voltage (pu)"
      mask help:
      | Notes:
      | Single Phase ZIP load model which gets converted to constant Z type if the voltage becomes lower than the Minimum Voltage.
      mask TypeOptions LoadType: Constant Z | constant I | constant P
      mask DialogControl ParameterTabVar0 Prompt: Parameters
      mask DialogControl ParameterTabVar1 Prompt: Type
      mask Display:
      | color('red');
      | A=[-210,-180,-170,-160,-147,-140,-130,-120,-110,-80,-50,-49,-45,-39,-33,-26,-21,-18,-17,-19,-22,-22,-26,-27,-25,-22,-16,-9,-3,2,6,6,4,1,1,-3,-4,-2,2,7,14,20,26,29,30,28,24,24,21,20,21,25,31,37,44,49,50,50,80];
      | B=[-41.5,-41.5,-63,-20,-63,-20,-63,-20,-41.5,-41.5,-41.5,-34,-26,-21,-20,-22,-28,-37,-47,-57,-63,-63,-54,-44,-34,-26,-21,-20,-22,-28,-37,-47,-57,-63,-63,-54,-44,-34,-26,-21,-20,-22,-28,-37,-47,-57,-63,-63,-54,-44,-34,-26,-21,-20,-22,-28,-37,-41.50,-41.5];
      | plot(A,B);
      | color('black');
      | port_label('LConn', 1, '+')
  55-56 1 : powerlib/Elements/Three-Phase PI Section Line  LConnTagsString=a|b|c  RConnTagsString=A|B|C  Frequency=60  Resistances=[R1_1 R0_1]  Inductances=[L1_1 L0_1]  Capacitances=[C1_1 C0_1]  Length=275*ft2km
      settings: SourceProductName=Simscape Electrical
  56 : powerlib/Measurements/Three-Phase V-I Measurement  VoltageMeasurement=phase-to-ground  SetLabelV=on  LabelV=V56  Vpu=off  VpuLL=off  CurrentMeasurement=no  SetLabelI=on  LabelI=I65  Ipu=off  Pbase=100e6  Vbase=24900  OutputType=Complex  PhasorSimulation=on  PSBequivalent=0
      settings: SourceProductName=Simscape Electrical
  56 Y PQ : Subsystem  mask(Single Phase ZIP Load){Vnom=1.0*2401.78, fnom=60, Pnom=20e3*a, Qnom=10e3*a, LoadType=constant P, Vlim=0.7}
      mask prompts: Vnom "Nominal Voltage Vn (Vrms)"; fnom "Nominal Frequency fn (Hz)"; Pnom "Nominal Active power (W)"; Qnom "Nominal Reactive power (VAR)"; LoadType "Load Type"; Vlim "Minimum voltage (pu)"
      mask help:
      | Notes:
      | Single Phase ZIP load model which gets converted to constant Z type if the voltage becomes lower than the Minimum Voltage.
      mask TypeOptions LoadType: Constant Z | constant I | constant P
      mask DialogControl ParameterTabVar0 Prompt: Parameters
      mask DialogControl ParameterTabVar1 Prompt: Type
      mask Display:
      | color('red');
      | A=[-210,-180,-170,-160,-147,-140,-130,-120,-110,-80,-50,-49,-45,-39,-33,-26,-21,-18,-17,-19,-22,-22,-26,-27,-25,-22,-16,-9,-3,2,6,6,4,1,1,-3,-4,-2,2,7,14,20,26,29,30,28,24,24,21,20,21,25,31,37,44,49,50,50,80];
      | B=[-41.5,-41.5,-63,-20,-63,-20,-63,-20,-41.5,-41.5,-41.5,-34,-26,-21,-20,-22,-28,-37,-47,-57,-63,-63,-54,-44,-34,-26,-21,-20,-22,-28,-37,-47,-57,-63,-63,-54,-44,-34,-26,-21,-20,-22,-28,-37,-47,-57,-63,-63,-54,-44,-34,-26,-21,-20,-22,-28,-37,-41.50,-41.5];
      | plot(A,B);
      | color('black');
      | port_label('LConn', 1, '+')
  57 : powerlib/Measurements/Three-Phase V-I Measurement  VoltageMeasurement=phase-to-ground  SetLabelV=on  LabelV=V57  Vpu=off  VpuLL=off  CurrentMeasurement=no  SetLabelI=on  LabelI=I65  Ipu=off  Pbase=100e6  Vbase=24900  OutputType=Complex  PhasorSimulation=on  PSBequivalent=0
      settings: SourceProductName=Simscape Electrical
  57-58 10 : powerlib/Elements/Pi Section Line  LConnTagsString=__new0  RConnTagsString=__new0  Frequency=60  Resistance=R1_10  Inductance=L1_10  Capacitance=C1_10  Length=250*ft2km  PiSections=1  Measurements=None
      settings: AttributesFormatString=\n  SourceProductName=Simscape Electrical  SourceProductBaseCode=PS
  57-60 3 : powerlib/Elements/Three-Phase PI Section Line  LConnTagsString=a|b|c  RConnTagsString=A|B|C  Frequency=60  Resistances=[R1_3 R0_3]  Inductances=[L1_3 L0_3]  Capacitances=[C1_3 C0_3]  Length=750*ft2km
      settings: SourceProductName=Simscape Electrical
  58 : Subsystem
  58 Y I : Subsystem  mask(Single Phase ZIP Load){Vnom=1.0*2401.78, fnom=60, Pnom=20e3*a, Qnom=10e3*a, LoadType=constant I, Vlim=0.7}
      mask prompts: Vnom "Nominal Voltage Vn (Vrms)"; fnom "Nominal Frequency fn (Hz)"; Pnom "Nominal Active power (W)"; Qnom "Nominal Reactive power (VAR)"; LoadType "Load Type"; Vlim "Minimum voltage (pu)"
      mask help:
      | Notes:
      | Single Phase ZIP load model which gets converted to constant Z type if the voltage becomes lower than the Minimum Voltage.
      mask TypeOptions LoadType: Constant Z | constant I | constant P
      mask DialogControl ParameterTabVar0 Prompt: Parameters
      mask DialogControl ParameterTabVar1 Prompt: Type
      mask Display:
      | color('red');
      | A=[-210,-180,-170,-160,-147,-140,-130,-120,-110,-80,-50,-49,-45,-39,-33,-26,-21,-18,-17,-19,-22,-22,-26,-27,-25,-22,-16,-9,-3,2,6,6,4,1,1,-3,-4,-2,2,7,14,20,26,29,30,28,24,24,21,20,21,25,31,37,44,49,50,50,80];
      | B=[-41.5,-41.5,-63,-20,-63,-20,-63,-20,-41.5,-41.5,-41.5,-34,-26,-21,-20,-22,-28,-37,-47,-57,-63,-63,-54,-44,-34,-26,-21,-20,-22,-28,-37,-47,-57,-63,-63,-54,-44,-34,-26,-21,-20,-22,-28,-37,-47,-57,-63,-63,-54,-44,-34,-26,-21,-20,-22,-28,-37,-41.50,-41.5];
      | plot(A,B);
      | color('black');
      | port_label('LConn', 1, '+')
  58-59 10 : powerlib/Elements/Pi Section Line  LConnTagsString=__new0  RConnTagsString=__new0  Frequency=60  Resistance=R1_10  Inductance=L1_10  Capacitance=C1_10  Length=10*ft2km  PiSections=1  Measurements=None
      settings: AttributesFormatString=\n  SourceProductName=Simscape Electrical  SourceProductBaseCode=PS
  59 : Subsystem
  59 Y PQ : Subsystem  mask(Single Phase ZIP Load){Vnom=1.0*2401.78, fnom=60, Pnom=20e3*a, Qnom=10e3*a, LoadType=constant P, Vlim=0.7}
      mask prompts: Vnom "Nominal Voltage Vn (Vrms)"; fnom "Nominal Frequency fn (Hz)"; Pnom "Nominal Active power (W)"; Qnom "Nominal Reactive power (VAR)"; LoadType "Load Type"; Vlim "Minimum voltage (pu)"
      mask help:
      | Notes:
      | Single Phase ZIP load model which gets converted to constant Z type if the voltage becomes lower than the Minimum Voltage.
      mask TypeOptions LoadType: Constant Z | constant I | constant P
      mask DialogControl ParameterTabVar0 Prompt: Parameters
      mask DialogControl ParameterTabVar1 Prompt: Type
      mask Display:
      | color('red');
      | A=[-210,-180,-170,-160,-147,-140,-130,-120,-110,-80,-50,-49,-45,-39,-33,-26,-21,-18,-17,-19,-22,-22,-26,-27,-25,-22,-16,-9,-3,2,6,6,4,1,1,-3,-4,-2,2,7,14,20,26,29,30,28,24,24,21,20,21,25,31,37,44,49,50,50,80];
      | B=[-41.5,-41.5,-63,-20,-63,-20,-63,-20,-41.5,-41.5,-41.5,-34,-26,-21,-20,-22,-28,-37,-47,-57,-63,-63,-54,-44,-34,-26,-21,-20,-22,-28,-37,-47,-57,-63,-63,-54,-44,-34,-26,-21,-20,-22,-28,-37,-47,-57,-63,-63,-54,-44,-34,-26,-21,-20,-22,-28,-37,-41.50,-41.5];
      | plot(A,B);
      | color('black');
      | port_label('LConn', 1, '+')
  59-94 : powerlib/Elements/Breaker  InitialState=0  SwitchingTimes="[1/60  5/60]"  External=off  BreakerResistance=0.01  SnubberResistance=1e6  SnubberCapacitance=inf  Measurements=None  MoreParameters=on  NoBreakLoop=off
      settings: SourceProductName=Simscape Electrical
  6 : Subsystem
  6 Y Z : Subsystem  mask(Single Phase ZIP Load){Vnom=1.0*2401.78, fnom=60, Pnom=40e3*a, Qnom=20e3*a, LoadType=Constant Z, Vlim=0.7}
      mask prompts: Vnom "Nominal Voltage Vn (Vrms)"; fnom "Nominal Frequency fn (Hz)"; Pnom "Nominal Active power (W)"; Qnom "Nominal Reactive power (VAR)"; LoadType "Load Type"; Vlim "Minimum voltage (pu)"
      mask help:
      | Notes:
      | Single Phase ZIP load model which gets converted to constant Z type if the voltage becomes lower than the Minimum Voltage.
      mask TypeOptions LoadType: Constant Z | constant I | constant P
      mask DialogControl ParameterTabVar0 Prompt: Parameters
      mask DialogControl ParameterTabVar1 Prompt: Type
      mask Display:
      | color('red');
      | A=[-210,-180,-170,-160,-147,-140,-130,-120,-110,-80,-50,-49,-45,-39,-33,-26,-21,-18,-17,-19,-22,-22,-26,-27,-25,-22,-16,-9,-3,2,6,6,4,1,1,-3,-4,-2,2,7,14,20,26,29,30,28,24,24,21,20,21,25,31,37,44,49,50,50,80];
      | B=[-41.5,-41.5,-63,-20,-63,-20,-63,-20,-41.5,-41.5,-41.5,-34,-26,-21,-20,-22,-28,-37,-47,-57,-63,-63,-54,-44,-34,-26,-21,-20,-22,-28,-37,-47,-57,-63,-63,-54,-44,-34,-26,-21,-20,-22,-28,-37,-47,-57,-63,-63,-54,-44,-34,-26,-21,-20,-22,-28,-37,-41.50,-41.5];
      | plot(A,B);
      | color('black');
      | port_label('LConn', 1, '+')
  60 : powerlib/Measurements/Three-Phase V-I Measurement  VoltageMeasurement=phase-to-ground  SetLabelV=on  LabelV=V60  Vpu=off  VpuLL=off  CurrentMeasurement=no  SetLabelI=on  LabelI=I65  Ipu=off  Pbase=100e6  Vbase=24900  OutputType=Complex  PhasorSimulation=on  PSBequivalent=0
      settings: SourceProductName=Simscape Electrical
  60 Y PQ : Subsystem  mask(Single Phase ZIP Load){Vnom=1.0*2401.78, fnom=60, Pnom=20e3*a, Qnom=10e3*a, LoadType=constant P, Vlim=0.7}
      mask prompts: Vnom "Nominal Voltage Vn (Vrms)"; fnom "Nominal Frequency fn (Hz)"; Pnom "Nominal Active power (W)"; Qnom "Nominal Reactive power (VAR)"; LoadType "Load Type"; Vlim "Minimum voltage (pu)"
      mask help:
      | Notes:
      | Single Phase ZIP load model which gets converted to constant Z type if the voltage becomes lower than the Minimum Voltage.
      mask TypeOptions LoadType: Constant Z | constant I | constant P
      mask DialogControl ParameterTabVar0 Prompt: Parameters
      mask DialogControl ParameterTabVar1 Prompt: Type
      mask Display:
      | color('red');
      | A=[-210,-180,-170,-160,-147,-140,-130,-120,-110,-80,-50,-49,-45,-39,-33,-26,-21,-18,-17,-19,-22,-22,-26,-27,-25,-22,-16,-9,-3,2,6,6,4,1,1,-3,-4,-2,2,7,14,20,26,29,30,28,24,24,21,20,21,25,31,37,44,49,50,50,80];
      | B=[-41.5,-41.5,-63,-20,-63,-20,-63,-20,-41.5,-41.5,-41.5,-34,-26,-21,-20,-22,-28,-37,-47,-57,-63,-63,-54,-44,-34,-26,-21,-20,-22,-28,-37,-47,-57,-63,-63,-54,-44,-34,-26,-21,-20,-22,-28,-37,-47,-57,-63,-63,-54,-44,-34,-26,-21,-20,-22,-28,-37,-41.50,-41.5];
      | plot(A,B);
      | color('black');
      | port_label('LConn', 1, '+')
  60-1 : powerlib/Elements/Three-Phase Breaker  InitialState=closed  SwitchA=off  SwitchB=off  SwitchC=off  SwitchTimes="[1/60  5/60]"  External=off  BreakerResistance=1e-6  SnubberResistance=1e6  SnubberCapacitance=inf  Measurements=None
      settings: SourceProductName=Simscape Electrical
  60-61 5 : powerlib/Elements/Three-Phase PI Section Line  LConnTagsString=a|b|c  RConnTagsString=A|B|C  Frequency=60  Resistances=[R1_5 R0_5]  Inductances=[L1_5 L0_5]  Capacitances=[C1_5 C0_5]  Length=550*ft2km
      settings: SourceProductName=Simscape Electrical
  60-62 12 : powerlib/Elements/Three-Phase PI Section Line  LConnTagsString=a|b|c  RConnTagsString=A|B|C  Frequency=60  Resistances=[R1_12 R0_12]  Inductances=[L1_12 L0_12]  Capacitances=[C1_12 C0_12]  Length=250*ft2km
      settings: SourceProductName=Simscape Electrical
  61 : powerlib/Measurements/Three-Phase V-I Measurement  VoltageMeasurement=phase-to-ground  SetLabelV=on  LabelV=V61  Vpu=off  VpuLL=off  CurrentMeasurement=no  SetLabelI=on  LabelI=I65  Ipu=off  Pbase=100e6  Vbase=24900  OutputType=Complex  PhasorSimulation=on  PSBequivalent=0
      settings: SourceProductName=Simscape Electrical
  61-610 : powerlib/Elements/Three-Phase Breaker  InitialState=closed  SwitchA=off  SwitchB=off  SwitchC=off  SwitchTimes="[1/60  5/60]"  External=off  BreakerResistance=1e-6  SnubberResistance=1e6  SnubberCapacitance=inf  Measurements=None
      settings: SourceProductName=Simscape Electrical
  610 : powerlib/Measurements/Three-Phase V-I Measurement  VoltageMeasurement=phase-to-phase  SetLabelV=on  LabelV=V610  Vpu=off  VpuLL=off  CurrentMeasurement=no  SetLabelI=on  LabelI=I65  Ipu=off  Pbase=100e6  Vbase=24900  OutputType=Complex  PhasorSimulation=on  PSBequivalent=0
      settings: SourceProductName=Simscape Electrical
  62 : powerlib/Measurements/Three-Phase V-I Measurement  VoltageMeasurement=phase-to-ground  SetLabelV=on  LabelV=V62  Vpu=off  VpuLL=off  CurrentMeasurement=no  SetLabelI=on  LabelI=I65  Ipu=off  Pbase=100e6  Vbase=24900  OutputType=Complex  PhasorSimulation=on  PSBequivalent=0
      settings: SourceProductName=Simscape Electrical
  62 Y Z : Subsystem  mask(Single Phase ZIP Load){Vnom=1.0*2401.78, fnom=60, Pnom=40e3*a, Qnom=20e3*a, LoadType=Constant Z, Vlim=0.7}
      mask prompts: Vnom "Nominal Voltage Vn (Vrms)"; fnom "Nominal Frequency fn (Hz)"; Pnom "Nominal Active power (W)"; Qnom "Nominal Reactive power (VAR)"; LoadType "Load Type"; Vlim "Minimum voltage (pu)"
      mask help:
      | Notes:
      | Single Phase ZIP load model which gets converted to constant Z type if the voltage becomes lower than the Minimum Voltage.
      mask TypeOptions LoadType: Constant Z | constant I | constant P
      mask DialogControl ParameterTabVar0 Prompt: Parameters
      mask DialogControl ParameterTabVar1 Prompt: Type
      mask Display:
      | color('red');
      | A=[-210,-180,-170,-160,-147,-140,-130,-120,-110,-80,-50,-49,-45,-39,-33,-26,-21,-18,-17,-19,-22,-22,-26,-27,-25,-22,-16,-9,-3,2,6,6,4,1,1,-3,-4,-2,2,7,14,20,26,29,30,28,24,24,21,20,21,25,31,37,44,49,50,50,80];
      | B=[-41.5,-41.5,-63,-20,-63,-20,-63,-20,-41.5,-41.5,-41.5,-34,-26,-21,-20,-22,-28,-37,-47,-57,-63,-63,-54,-44,-34,-26,-21,-20,-22,-28,-37,-47,-57,-63,-63,-54,-44,-34,-26,-21,-20,-22,-28,-37,-47,-57,-63,-63,-54,-44,-34,-26,-21,-20,-22,-28,-37,-41.50,-41.5];
      | plot(A,B);
      | color('black');
      | port_label('LConn', 1, '+')
  62-63 12 : powerlib/Elements/Three-Phase PI Section Line  LConnTagsString=a|b|c  RConnTagsString=A|B|C  Frequency=60  Resistances=[R1_12 R0_12]  Inductances=[L1_12 L0_12]  Capacitances=[C1_12 C0_12]  Length=175*ft2km
      settings: SourceProductName=Simscape Electrical
  63 : powerlib/Measurements/Three-Phase V-I Measurement  VoltageMeasurement=phase-to-ground  SetLabelV=on  LabelV=V63  Vpu=off  VpuLL=off  CurrentMeasurement=no  SetLabelI=on  LabelI=I65  Ipu=off  Pbase=100e6  Vbase=24900  OutputType=Complex  PhasorSimulation=on  PSBequivalent=0
      settings: SourceProductName=Simscape Electrical
  63 Y PQ : Subsystem  mask(Single Phase ZIP Load){Vnom=1.0*2401.78, fnom=60, Pnom=40e3*a, Qnom=20e3*a, LoadType=constant P, Vlim=0.7}
      mask prompts: Vnom "Nominal Voltage Vn (Vrms)"; fnom "Nominal Frequency fn (Hz)"; Pnom "Nominal Active power (W)"; Qnom "Nominal Reactive power (VAR)"; LoadType "Load Type"; Vlim "Minimum voltage (pu)"
      mask help:
      | Notes:
      | Single Phase ZIP load model which gets converted to constant Z type if the voltage becomes lower than the Minimum Voltage.
      mask TypeOptions LoadType: Constant Z | constant I | constant P
      mask DialogControl ParameterTabVar0 Prompt: Parameters
      mask DialogControl ParameterTabVar1 Prompt: Type
      mask Display:
      | color('red');
      | A=[-210,-180,-170,-160,-147,-140,-130,-120,-110,-80,-50,-49,-45,-39,-33,-26,-21,-18,-17,-19,-22,-22,-26,-27,-25,-22,-16,-9,-3,2,6,6,4,1,1,-3,-4,-2,2,7,14,20,26,29,30,28,24,24,21,20,21,25,31,37,44,49,50,50,80];
      | B=[-41.5,-41.5,-63,-20,-63,-20,-63,-20,-41.5,-41.5,-41.5,-34,-26,-21,-20,-22,-28,-37,-47,-57,-63,-63,-54,-44,-34,-26,-21,-20,-22,-28,-37,-47,-57,-63,-63,-54,-44,-34,-26,-21,-20,-22,-28,-37,-47,-57,-63,-63,-54,-44,-34,-26,-21,-20,-22,-28,-37,-41.50,-41.5];
      | plot(A,B);
      | color('black');
      | port_label('LConn', 1, '+')
  63-64 12 : powerlib/Elements/Three-Phase PI Section Line  LConnTagsString=a|b|c  RConnTagsString=A|B|C  Frequency=60  Resistances=[R1_12 R0_12]  Inductances=[L1_12 L0_12]  Capacitances=[C1_12 C0_12]  Length=350*ft2km
      settings: SourceProductName=Simscape Electrical
  64 : powerlib/Measurements/Three-Phase V-I Measurement  VoltageMeasurement=phase-to-ground  SetLabelV=on  LabelV=V64  Vpu=off  VpuLL=off  CurrentMeasurement=no  SetLabelI=on  LabelI=I65  Ipu=off  Pbase=100e6  Vbase=24900  OutputType=Complex  PhasorSimulation=on  PSBequivalent=0
      settings: SourceProductName=Simscape Electrical
  64 Y I : Subsystem  mask(Single Phase ZIP Load){Vnom=1.0*2401.78, fnom=60, Pnom=75e3*a, Qnom=35e3*a, LoadType=constant I, Vlim=0.7}
      mask prompts: Vnom "Nominal Voltage Vn (Vrms)"; fnom "Nominal Frequency fn (Hz)"; Pnom "Nominal Active power (W)"; Qnom "Nominal Reactive power (VAR)"; LoadType "Load Type"; Vlim "Minimum voltage (pu)"
      mask help:
      | Notes:
      | Single Phase ZIP load model which gets converted to constant Z type if the voltage becomes lower than the Minimum Voltage.
      mask TypeOptions LoadType: Constant Z | constant I | constant P
      mask DialogControl ParameterTabVar0 Prompt: Parameters
      mask DialogControl ParameterTabVar1 Prompt: Type
      mask Display:
      | color('red');
      | A=[-210,-180,-170,-160,-147,-140,-130,-120,-110,-80,-50,-49,-45,-39,-33,-26,-21,-18,-17,-19,-22,-22,-26,-27,-25,-22,-16,-9,-3,2,6,6,4,1,1,-3,-4,-2,2,7,14,20,26,29,30,28,24,24,21,20,21,25,31,37,44,49,50,50,80];
      | B=[-41.5,-41.5,-63,-20,-63,-20,-63,-20,-41.5,-41.5,-41.5,-34,-26,-21,-20,-22,-28,-37,-47,-57,-63,-63,-54,-44,-34,-26,-21,-20,-22,-28,-37,-47,-57,-63,-63,-54,-44,-34,-26,-21,-20,-22,-28,-37,-47,-57,-63,-63,-54,-44,-34,-26,-21,-20,-22,-28,-37,-41.50,-41.5];
      | plot(A,B);
      | color('black');
      | port_label('LConn', 1, '+')
  64-65 12 : powerlib/Elements/Three-Phase PI Section Line  LConnTagsString=a|b|c  RConnTagsString=A|B|C  Frequency=60  Resistances=[R1_12 R0_12]  Inductances=[L1_12 L0_12]  Capacitances=[C1_12 C0_12]  Length=425*ft2km
      settings: SourceProductName=Simscape Electrical
  65 : powerlib/Measurements/Three-Phase V-I Measurement  VoltageMeasurement=phase-to-ground  SetLabelV=on  LabelV=V65  Vpu=off  VpuLL=off  CurrentMeasurement=yes  SetLabelI=on  LabelI=I65  Ipu=off  Pbase=100e6  Vbase=24900  OutputType=Complex  PhasorSimulation=on  PSBequivalent=0
      settings: SourceProductName=Simscape Electrical
  65 D Z : Subsystem  mask(Three Phase Delta ZIP Load (Phasor)){Vnom=4160, fnom=60, Pnom=[35 35 70]*1e3*a, Qnom=[25 25 50]*1e3*a, LoadType=Constant Z, Vlim=0.7}
      mask prompts: Vnom "Nominal Ph-Ph Voltage (Vrms)"; fnom "Nominal Frequency fn (Hz)"; Pnom "Nominal Per Phase Active Power [Pab Pbc Pca] (W)"; Qnom "Nominal Per Phase Reactive Power [Qab Qbc Qca] (VAR)"; LoadType "Load Type"; Vlim "Minimum Voltage (pu)"
      mask help:
      | Notes:
      | Three Phase Delta Connected ZIP load model which gets converted to constant Z type if the voltage becomes lower than the Minimum Voltage.
      mask TypeOptions LoadType: Constant Z | Constant I | Constant P
      mask DialogControl ParameterTabVar0 Prompt: Parameters
      mask DialogControl ParameterTabVar01 Prompt: Type
      mask Display:
      | color('red');
      | %load figure 0deg
      | A=[-210,-180,-170,-160,-147,-140,-130,-120,-110,-80,-50,-49,-45,-39,-33,-26,-21,-18,-17,-19,-22,-22,-26,-27,-25,-22,-16,-9,-3,2,6,6,4,1,1,-3,-4,-2,2,7,14,20,26,29,30,28,24,24,21,20,21,25,31,37,44,49,50,50,80];
      | B=[-41.5,-41.5,-63,-20,-63,-20,-63,-20,-41.5,-41.5,-41.5,-34,-26,-21,-20,-22,-28,-37,-47,-57,-63,-63,-54,-44,-34,-26,-21,-20,-22,-28,-37,-47,-57,-63,-63,-54,-44,-34,-26,-21,-20,-22,-28,-37,-47,-57,-63,-63,-54,-44,-34,-26,-21,-20,-22,-28,-37,-41.50,-41.5];
      | plot(A,B);
      | 
      | %load figure 0deg inverted
      | A1=[-80,-50,-49,-45,-39,-33,-26,-21,-18,-17,-19,-22,-22,-26,-27,-25,-22,-16,-9,-3,2,6,6,4,1,1,-3,-4,-2,2,7,14,20,26,29,30,28,24,24,21,20,21,25,31,37,44,49,50,50,80,110,120,130,143,150,160,170,180,210];
      | B1=[-41.5,-41.5,-34,-26,-21,-20,-22,-28,-37,-47,-57,-63,-63,-54,-44,-34,-26,-21,-20,-22,-28,-37,-47,-57,-63,-63,-54,-44,-34,-26,-21,-20,-22,-28,-37,-47,-57,-63,-63,-54,-44,-34,-26,-21,-20,-22,-28,-37,-41.5,-41.5,-41.5,-63,-20,-63,-20,-63,-20,-41.5,-41.5];
      | 
      | 
      | %load figure -120deg
      | c=1*exp(sqrt(-1)*(-60*pi/180));
      | l=A1+j*B1;
      | m=l*c;
      | E=real(m);F=imag(m);
      | E=E+10.94;F=F+161.1;
      | plot(E,F);
      | 
      | %load figure +120deg
      | c=1*exp(sqrt(-1)*(60*pi/180));
      | l=A1+j*B1;
      | m=l*c;
      | G=real(m);
      | H=imag(m);
      | G=G-205.94;H=H+48.53;
      | plot(G,H);
      | 
      | color('black');
      | port_label('LConn', 1, 'A')
      | port_label('LConn', 2, 'B')
      | port_label('LConn', 3, 'C')
  65-66 12 : powerlib/Elements/Three-Phase PI Section Line  LConnTagsString=a|b|c  RConnTagsString=A|B|C  Frequency=60  Resistances=[R1_12 R0_12]  Inductances=[L1_12 L0_12]  Capacitances=[C1_12 C0_12]  Length=325*ft2km
      settings: SourceProductName=Simscape Electrical
  66 : powerlib/Measurements/Three-Phase V-I Measurement  VoltageMeasurement=phase-to-ground  SetLabelV=on  LabelV=V66  Vpu=off  VpuLL=off  CurrentMeasurement=no  SetLabelI=on  LabelI=I65  Ipu=off  Pbase=100e6  Vbase=24900  OutputType=Complex  PhasorSimulation=on  PSBequivalent=0
      settings: SourceProductName=Simscape Electrical
  66 Y PQ : Subsystem  mask(Single Phase ZIP Load){Vnom=1.0*2401.78, fnom=60, Pnom=75e3*a, Qnom=35e3*a, LoadType=constant P, Vlim=0.7}
      mask prompts: Vnom "Nominal Voltage Vn (Vrms)"; fnom "Nominal Frequency fn (Hz)"; Pnom "Nominal Active power (W)"; Qnom "Nominal Reactive power (VAR)"; LoadType "Load Type"; Vlim "Minimum voltage (pu)"
      mask help:
      | Notes:
      | Single Phase ZIP load model which gets converted to constant Z type if the voltage becomes lower than the Minimum Voltage.
      mask TypeOptions LoadType: Constant Z | constant I | constant P
      mask DialogControl ParameterTabVar0 Prompt: Parameters
      mask DialogControl ParameterTabVar1 Prompt: Type
      mask Display:
      | color('red');
      | A=[-210,-180,-170,-160,-147,-140,-130,-120,-110,-80,-50,-49,-45,-39,-33,-26,-21,-18,-17,-19,-22,-22,-26,-27,-25,-22,-16,-9,-3,2,6,6,4,1,1,-3,-4,-2,2,7,14,20,26,29,30,28,24,24,21,20,21,25,31,37,44,49,50,50,80];
      | B=[-41.5,-41.5,-63,-20,-63,-20,-63,-20,-41.5,-41.5,-41.5,-34,-26,-21,-20,-22,-28,-37,-47,-57,-63,-63,-54,-44,-34,-26,-21,-20,-22,-28,-37,-47,-57,-63,-63,-54,-44,-34,-26,-21,-20,-22,-28,-37,-47,-57,-63,-63,-54,-44,-34,-26,-21,-20,-22,-28,-37,-41.50,-41.5];
      | plot(A,B);
      | color('black');
      | port_label('LConn', 1, '+')
  67 : powerlib/Measurements/Three-Phase V-I Measurement  VoltageMeasurement=phase-to-ground  SetLabelV=on  LabelV=V67  Vpu=off  VpuLL=off  CurrentMeasurement=no  SetLabelI=on  LabelI=I65  Ipu=off  Pbase=100e6  Vbase=24900  OutputType=Complex  PhasorSimulation=on  PSBequivalent=0
      settings: SourceProductName=Simscape Electrical
  67-68 9 : powerlib/Elements/Pi Section Line  LConnTagsString=__new0  RConnTagsString=__new0  Frequency=60  Resistance=R1_9  Inductance=L1_9  Capacitance=C1_9  Length=200*ft2km  PiSections=1  Measurements=None
      settings: AttributesFormatString=\n  SourceProductName=Simscape Electrical  SourceProductBaseCode=PS
  67-72 3 : powerlib/Elements/Three-Phase PI Section Line  LConnTagsString=a|b|c  RConnTagsString=A|B|C  Frequency=60  Resistances=[R1_3 R0_3]  Inductances=[L1_3 L0_3]  Capacitances=[C1_3 C0_3]  Length=275*ft2km
      settings: SourceProductName=Simscape Electrical
  67-97 3 : Subsystem  mask(Three-Phase PI Section Block){Rl=R_3, Ll=L_3, Cl=C_3, L=350*ft2km}
      mask prompts: Rl "Resistance per unit Length(Ohm/Km)[3x3 matrix]"; Ll "Inductance per unit Length(H/Km)[3x3 matrix]"; Cl "Capacitance per unit Length(F/Km)[3x3 matrix]"; L "Length (Km)"
      mask help: This block models a three-phase transmission line with a single PI section.
  68 : Subsystem
  68 Y PQ : Subsystem  mask(Single Phase ZIP Load){Vnom=1.0*2401.78, fnom=60, Pnom=20e3*a, Qnom=10e3*a, LoadType=constant P, Vlim=0.7}
      mask prompts: Vnom "Nominal Voltage Vn (Vrms)"; fnom "Nominal Frequency fn (Hz)"; Pnom "Nominal Active power (W)"; Qnom "Nominal Reactive power (VAR)"; LoadType "Load Type"; Vlim "Minimum voltage (pu)"
      mask help:
      | Notes:
      | Single Phase ZIP load model which gets converted to constant Z type if the voltage becomes lower than the Minimum Voltage.
      mask TypeOptions LoadType: Constant Z | constant I | constant P
      mask DialogControl ParameterTabVar0 Prompt: Parameters
      mask DialogControl ParameterTabVar1 Prompt: Type
      mask Display:
      | color('red');
      | A=[-210,-180,-170,-160,-147,-140,-130,-120,-110,-80,-50,-49,-45,-39,-33,-26,-21,-18,-17,-19,-22,-22,-26,-27,-25,-22,-16,-9,-3,2,6,6,4,1,1,-3,-4,-2,2,7,14,20,26,29,30,28,24,24,21,20,21,25,31,37,44,49,50,50,80];
      | B=[-41.5,-41.5,-63,-20,-63,-20,-63,-20,-41.5,-41.5,-41.5,-34,-26,-21,-20,-22,-28,-37,-47,-57,-63,-63,-54,-44,-34,-26,-21,-20,-22,-28,-37,-47,-57,-63,-63,-54,-44,-34,-26,-21,-20,-22,-28,-37,-47,-57,-63,-63,-54,-44,-34,-26,-21,-20,-22,-28,-37,-41.50,-41.5];
      | plot(A,B);
      | color('black');
      | port_label('LConn', 1, '+')
  68-69 9 : powerlib/Elements/Pi Section Line  LConnTagsString=__new0  RConnTagsString=__new0  Frequency=60  Resistance=R1_9  Inductance=L1_9  Capacitance=C1_9  Length=275*ft2km  PiSections=1  Measurements=None
      settings: AttributesFormatString=\n  SourceProductName=Simscape Electrical  SourceProductBaseCode=PS
  69 : Subsystem
  69 Y PQ : Subsystem  mask(Single Phase ZIP Load){Vnom=1.0*2401.78, fnom=60, Pnom=40e3*a, Qnom=20e3*a, LoadType=constant P, Vlim=0.7}
      mask prompts: Vnom "Nominal Voltage Vn (Vrms)"; fnom "Nominal Frequency fn (Hz)"; Pnom "Nominal Active power (W)"; Qnom "Nominal Reactive power (VAR)"; LoadType "Load Type"; Vlim "Minimum voltage (pu)"
      mask help:
      | Notes:
      | Single Phase ZIP load model which gets converted to constant Z type if the voltage becomes lower than the Minimum Voltage.
      mask TypeOptions LoadType: Constant Z | constant I | constant P
      mask DialogControl ParameterTabVar0 Prompt: Parameters
      mask DialogControl ParameterTabVar1 Prompt: Type
      mask Display:
      | color('red');
      | A=[-210,-180,-170,-160,-147,-140,-130,-120,-110,-80,-50,-49,-45,-39,-33,-26,-21,-18,-17,-19,-22,-22,-26,-27,-25,-22,-16,-9,-3,2,6,6,4,1,1,-3,-4,-2,2,7,14,20,26,29,30,28,24,24,21,20,21,25,31,37,44,49,50,50,80];
      | B=[-41.5,-41.5,-63,-20,-63,-20,-63,-20,-41.5,-41.5,-41.5,-34,-26,-21,-20,-22,-28,-37,-47,-57,-63,-63,-54,-44,-34,-26,-21,-20,-22,-28,-37,-47,-57,-63,-63,-54,-44,-34,-26,-21,-20,-22,-28,-37,-47,-57,-63,-63,-54,-44,-34,-26,-21,-20,-22,-28,-37,-41.50,-41.5];
      | plot(A,B);
      | color('black');
      | port_label('LConn', 1, '+')
  69-70 9 : powerlib/Elements/Pi Section Line  LConnTagsString=__new0  RConnTagsString=__new0  Frequency=60  Resistance=R1_9  Inductance=L1_9  Capacitance=C1_9  Length=325*ft2km  PiSections=1  Measurements=None
      settings: AttributesFormatString=\n  SourceProductName=Simscape Electrical  SourceProductBaseCode=PS
  7 : powerlib/Measurements/Three-Phase V-I Measurement  VoltageMeasurement=phase-to-ground  SetLabelV=on  LabelV=V7  Vpu=off  VpuLL=off  CurrentMeasurement=no  SetLabelI=on  LabelI=I800  Ipu=off  Pbase=100e6  Vbase=24900  OutputType=Complex  PhasorSimulation=on  PSBequivalent=0
      settings: SourceProductName=Simscape Electrical
  7 Y PQ : Subsystem  mask(Single Phase ZIP Load){Vnom=1.0*2401.78, fnom=60, Pnom=20e3*a, Qnom=10e3*a, LoadType=constant P, Vlim=0.7}
      mask prompts: Vnom "Nominal Voltage Vn (Vrms)"; fnom "Nominal Frequency fn (Hz)"; Pnom "Nominal Active power (W)"; Qnom "Nominal Reactive power (VAR)"; LoadType "Load Type"; Vlim "Minimum voltage (pu)"
      mask help:
      | Notes:
      | Single Phase ZIP load model which gets converted to constant Z type if the voltage becomes lower than the Minimum Voltage.
      mask TypeOptions LoadType: Constant Z | constant I | constant P
      mask DialogControl ParameterTabVar0 Prompt: Parameters
      mask DialogControl ParameterTabVar1 Prompt: Type
      mask Display:
      | color('red');
      | A=[-210,-180,-170,-160,-147,-140,-130,-120,-110,-80,-50,-49,-45,-39,-33,-26,-21,-18,-17,-19,-22,-22,-26,-27,-25,-22,-16,-9,-3,2,6,6,4,1,1,-3,-4,-2,2,7,14,20,26,29,30,28,24,24,21,20,21,25,31,37,44,49,50,50,80];
      | B=[-41.5,-41.5,-63,-20,-63,-20,-63,-20,-41.5,-41.5,-41.5,-34,-26,-21,-20,-22,-28,-37,-47,-57,-63,-63,-54,-44,-34,-26,-21,-20,-22,-28,-37,-47,-57,-63,-63,-54,-44,-34,-26,-21,-20,-22,-28,-37,-47,-57,-63,-63,-54,-44,-34,-26,-21,-20,-22,-28,-37,-41.50,-41.5];
      | plot(A,B);
      | color('black');
      | port_label('LConn', 1, '+')
  7-8 1 : powerlib/Elements/Three-Phase PI Section Line  LConnTagsString=a|b|c  RConnTagsString=A|B|C  Frequency=60  Resistances=[R1_1 R0_1]  Inductances=[L1_1 L0_1]  Capacitances=[C1_1 C0_1]  Length=200*ft2km
      settings: SourceProductName=Simscape Electrical
  70 : Subsystem
